simulink model "abslut125_fixpt16"  (R2021b)
(part 3 of 8)

  ROM6 : hdlBasic/ROM  depth=7874  initVector=[1,0,0,0,0,1,0,1,1,1,1,1,1,0,0,1,1,0,0,1,1,1,0,0,1,1,1,0,0,0,0,1,1,0,0,0,0,0,1,1,0,0,0,1,1,0,1,1,0,0,0,1,1,1,0,1,1,0,0,0,1,1,1,0,0,1,1,1,0,0,1,1,1,0,0,1,1,1,1,0,0,1,1,1,0,0,1,1,1,0,0,0,0,1,1,1,0,0,0,1,1,0,0,0,1,0,0,1,1,0,0,0,1,1,0,0,0,1,1,1,0,1,1,0,0,0,1,1,0,0,0,1,1,1,0,0,1,1,1,0,0,1,1,1,0,0,1,1,1,0,0,1,1,1,1,0,0,1,1,1,0,0,1,1,1,0,0,1,1,1,0,1,0,0,1,1,1,0,0,1,1,1,0,0,1,1,1,0,0,0,0,0,0,1,1,0,0,0,1,1,0,0,0,1,1,0,0,0,1,1,0,0,1,1,0,0,0,1,1,0,0,0,1,1,0,0,0,1,1,1,0,0,1,1,1,0,0,1,1,0,0,0,1,1,0,0,0,1,1,1,0,0,1,0,1,1,0,0,1,1,1,0,0,1,1,1,0,0,1,1,1,0,0,1,1,1,1,1,0,0,0,1,1,0,0,1,1,1,0,0,1,1,1,0,0,1,1,1,0,0,1,1,0,0,1,1,0,0,0,1,1,0,0,0,1,1,0,0,0,1,1,0,0,0,1,1,0,0,1,1,1,0,0,1,1,0,0,0,1,1,0,0,0,1,1,0,0,0,1,1,1,1,0,0,1,1,0,0,1,1,1,0,0,1,1,0,0,0,1,1,0,0,0,1,1,1,0,0,0,0,1,1,0,0,0,1,1,0,0,1,1,1,0,0,1,1,1,0,0,1,1,1,0,0,1,1,0,0,1,1,0,0,1,1,0,0,0,1,1,0,0,1,1,1,0,0,1,1,1,0,0,1,1,1,0,0,1,1,0,0,1,1,1,0,0,1,1,0,0,0,1,1,0,0,1,1,1,0,0,1,1,1,0,0,0,0,1,1,0,0,1,1,0,0,1,1,1,0,0,1,1,0,0,0,1,1,0,0,0,1,1,0,0,0,1,1,1,1,0,0,1,1,1,0,0,1,1,0,0,1,1,1,0,0,1,1,0,0,0,1,1,0,0,0,1,1,0,0,1,1,0,0,1,1,0,0,1,1,0,0,0,1,1,0,0,1,1,1,0,0,1,1,0,0,0,1,1,1,0,0,1,1,0,0,1,1,1,0,0,1,1,0,0,1,1,0,0,0,1,1,0,0,1,1,1,0,0,1,1,1,0,0,1,1,1,1,0,0,1,1,0,0,1,1,0,0,0,1,1,0,0,1,1,0,0,0,1,1,0,0,1,1,1,0,0,1,1,1,0,0,0,0,1,1,1,0,0,1,1,0,0,1,1,0,0,1,1,1,0,0,1,1,0,0,0,1,1,0,0,0,1,1,0,0,0,1,0,0,1,1,0,0,1,1,0,0,0,1,1,0,0,1,1,0,0,1,1,1,0,0,1,1,0,0,0,1,1,0,0,0,1,1,0,0,0,1,1,0,0,1,1,0,0,1,1,0,0,1,1,1,0,0,1,1,0,0,1,1,1,0,0,1,1,0,0,0,1,1,0,0,0,0,1,1,0,0,1,1,0,0,0,1,1,0,0,1,1,0,0,1,1,0,0,0,1,1,0,0,1,1,1,0,0,1,1,1,0,0,1,1,0,1,1,0,0,1,1,0,0,1,1,0,0,1,1,1,0,0,1,1,0,0,1,1,0,0,0,1,1,0,0,1,1,1,0,0,1,1,1,0,1,1,0,0,0,1,1,0,0,1,1,0,0,1,1,0,0,1,1,0,0,0,1,1,0,0,1,1,0,0,0,1,1,0,0,1,1,1,0,0,0,1,1,0,0,1,1,0,0,1,1,0,0,1,1,1,0,0,1,1,0,0,1,1,0,0,1,1,1,0,0,1,1,0,0,0,1,1,0,0,0,1,1,1,1,0,0,1,1,0,0,1,1,0,0,1,1,0,0,1,1,0,0,0,1,1,0,0,1,1,0,0,1,1,1,0,0,1,1,0,0,0,1,1,0,0,1,0,0,1,1,1,0,0,1,1,0,0,1,1,0,0,1,1,0,0,1,1,0,0,1,1,1,0,0,1,1,0,0,1,1,1,0,0,1,1,1,0,0,1,1,0,0,1,1,0,0,1,1,0,0,1,1,0,0,1,1,1,0,0,1,1,0,0,1,1,0,0,1,1,0,0,0,1,1,0,0,1,1,1,0,0,1,1,1,1,0,0,1,1,0,0,1,1,0,0,1,1,0,0,1,1,0,0,1,1,0,0,1,1,1,0,0,1,1,0,0,1,1,0,0,0,1,1,0,0,1,1,1,0,0,1,0,0,1,1,0,0,1,1,0,0,1,1,0,0,1,1,0,0,1,1,0,0,1,1,0,0,1,1,0,0,0,1,1,0,0,1,1,0,0,0,1,1,0,0,0,1,0,0,1,1,0,0,1,1,0,0,1,1,0,0,1,1,0,0,1,1,1,0,0,1,1,0,0,1,1,0,0,1,1,0,0,1,1,1,0,0,1,1,0,0,0,1,1,0,0,0,1,1,0,0,1,1,0,0,1,1,0,0,1,1,0,0,1,1,0,0,1,1,0,0,1,1,0,0,0,1,1,0,0,1,1,0,0,1,1,1,0,0,1,1,0,0,0,0,0,1,1,0,0,1,1,0,0,1,1,0,0,1,1,0,0,1,1,0,0,1,1,0,0,1,1,0,0,1,1,0,0,1,1,1,0,0,1,1,0,0,1,1,1,0,0,1,1,0,0,1,1,0,0,1,1,0,0,1,1,0,0,1,1,0,0,1,1,0,0,1,1,0,0,1,1,0,0,1,1,0,0,1,1,0,0,1,1,0,0,0,1,1,0,0,1,1,1,0,0,1,1,0,0,1,1,0,0,1,1,0,0,1,1,0,0,1,1,0,0,1,1,0,0,1,1,0,0,1,1,0,0,0,1,1,0,0,1,1,0,0,1,1,0,0,0,1,1,0,0,0,0,1,1,0,0,1,1,0,0,1,1,0,0,1,1,0,0,1,1,0,0,1,1,0,0,1,1,0,0,1,1,0,0,1,1,0,0,1,1,0,0,0,1,1,0,0,1,1,0,0,0,1,1,0,1,1,0,0,1,1,0,0,1,1,0,0,1,1,0,0,1,1,0,0,1,1,0,0,1,1,0,0,1,1,0,0,1,1,0,0,1,1,0,0,1,1,0,0,1,1,1,0,0,1,1,0,0,0,1,1,0,0,1,1,0,0,1,1,0,0,1,1,0,0,1,1,0,0,1,1,0,0,1,1,0,0,1,1,0,0,1,1,0,0,1,1,0,0,1,1,0,0,1,1,0,0,1,1,1,0,0,1,0,1,1,0,0,1,1,0,0,1,1,0,0,1,1,0,0,1,0,0,1,1,0,0,1,1,0,0,1,1,0,0,1,1,0,0,1,1,0,0,1,1,0,0,1,1,1,0,0,1,1,0,0,1,1,1,0,1,1,0,0,1,1,0,0,1,1,0,1,1,0,0,1,1,0,0,1,1,0,0,1,1,0,0,1,1,0,0,1,1,0,0,1,1,0,0,1,1,0,0,1,1,0,0,1,1,0,0,0,1,1,0,0,0,1,1,0,0,1,1,0,1,1,0,0,1,1,0,0,1,1,0,0,1,1,0,0,1,1,0,0,1,1,0,0,1,1,0,0,1,1,0,0,1,1,0,0,1,1,0,0,1,1,0,0,1,1,0,0,0,1,0,1,1,0,0,1,0,0,1,1,0,0,1,1,0,0,1,1,0,0,1,1,0,0,1,1,0,0,1,1,0,0,1,1,0,0,1,1,0,0,1,1,0,0,1,1,0,0,1,1,0,0,1,1,0,0,1,1,0,0,1,1,0,1,1,0,0,1,1,0,0,1,1,0,0,1,1,0,0,1,1,0,0,1,1,0,0,1,1,0,0,1,1,0,0,1,0,0,1,1,0,0,1,1,0,0,1,1,0,0,1,1,0,0,1,1,1,0,0,0,1,0,0,1,1,0,0,1,1,0,0,1,1,0,0,1,1,0,0,1,1,0,0,1,1,0,0,1,1,0,0,1,1,0,1,1,0,0,1,1,0,0,1,1,0,0,1,1,0,0,1,1,0,0,1,1,0,0,1,1,0,1,0,0,1,1,0,0,1,1,0,0,1,1,0,0,1,1,0,0,1,1,0,0,1,1,0,0,1,1,0,0,1,0,0,1,1,0,0,1,1,0,0,1,1,0,0,1,1,0,0,1,1,0,0,1,1,0,0,1,1,0,0,1,0,0,1,1,0,0,1,1,0,0,1,1,0,0,1,1,0,0,1,1,0,0,1,1,0,0,1,1,0,0,1,0,0,1,1,0,0,1,1,0,0,1,1,0 ...(+11750 chars)]  distributed_mem=Block RAM  rst=off  init_reg=0  en=off  latency=1  gui_display_data_type=Boolean  arith_type=Boolean  n_bits=2  bin_pt=0  preci_type=Double  exp_width=8  frac_width=24  optimize=Area  use_rpm=on  simulation_type=fast_sim  XmcBlockStatus=1  maskContainerNames=tabcontainer1  block_type=sprom  block_config=sysgen:SPROM_config
  ROM7 : hdlBasic/ROM  depth=7874  initVector=[0,1,1,1,0,1,0,1,0,0,1,0,0,1,0,0,0,1,0,1,1,0,1,0,1,1,0,1,1,0,0,1,0,1,1,0,0,0,1,0,1,1,0,1,0,0,1,0,1,1,0,1,0,0,1,1,0,1,1,0,1,0,0,1,0,1,0,0,1,0,1,0,0,1,0,1,1,0,0,1,0,1,1,0,1,0,1,1,0,1,0,1,0,1,1,0,1,0,0,1,0,1,1,0,1,0,0,1,0,1,0,0,1,0,1,1,0,1,0,0,0,1,0,1,1,0,1,0,1,1,0,1,0,0,1,0,1,0,0,1,0,1,0,0,1,0,1,0,0,1,0,1,1,1,0,1,0,1,0,0,1,0,1,0,0,1,0,1,1,0,1,0,1,0,1,1,0,1,0,1,1,0,1,0,1,1,0,1,0,0,1,1,0,1,0,1,0,0,1,0,1,0,0,1,0,1,0,0,1,0,1,0,1,0,1,1,0,1,0,1,0,0,1,0,1,1,0,1,0,0,1,0,1,1,0,1,0,1,0,1,1,0,1,0,1,1,0,1,0,0,1,0,1,0,1,0,1,0,1,1,0,1,0,1,0,0,1,0,1,0,0,1,0,1,1,0,1,0,1,1,0,1,0,1,0,1,1,0,1,0,1,1,0,1,0,1,1,0,1,0,1,0,1,0,1,0,1,1,0,1,0,1,0,0,1,0,1,0,0,1,0,1,0,0,1,0,1,0,1,1,0,1,0,1,0,1,1,0,1,0,1,0,0,1,0,1,1,0,1,0,0,0,1,0,1,0,1,0,1,0,0,1,0,1,0,1,1,0,1,0,1,1,0,1,0,0,1,0,1,0,1,0,1,1,0,1,0,1,0,1,1,0,1,0,1,0,0,1,0,1,0,0,1,0,1,1,0,0,1,0,1,0,1,0,1,0,0,1,0,1,0,1,1,0,1,0,1,0,0,1,0,1,1,0,1,0,1,0,1,0,1,1,0,1,0,1,0,1,0,0,1,0,1,0,1,1,0,1,0,1,1,0,1,0,0,0,1,0,1,0,1,0,1,0,1,1,0,1,0,1,0,1,0,0,1,0,1,0,0,1,0,1,0,0,1,0,1,0,1,0,1,0,0,1,0,1,0,1,0,1,0,0,1,0,1,0,1,1,0,1,0,1,1,0,1,0,1,1,1,0,1,0,1,0,1,0,1,0,1,1,0,1,0,1,0,1,0,0,1,0,1,0,1,1,0,1,0,0,1,0,1,0,1,0,1,0,0,1,0,1,0,1,0,1,0,1,1,0,1,0,1,0,1,1,0,1,0,1,0,0,1,0,1,1,0,0,1,0,1,0,1,0,1,0,1,0,0,1,0,1,0,1,0,1,0,0,1,0,1,0,1,1,0,1,0,1,1,0,1,0,1,0,1,0,0,1,0,1,0,1,0,1,0,1,0,1,1,0,1,0,1,0,1,0,0,1,0,1,0,0,1,0,1,0,0,1,1,0,1,0,1,0,1,0,1,0,0,1,0,1,0,1,0,1,0,1,0,0,1,0,1,0,1,1,0,1,0,1,0,0,1,0,1,1,0,1,0,1,0,1,0,1,0,1,0,1,0,1,0,0,1,0,1,0,1,0,1,0,0,1,0,1,0,1,1,0,1,0,1,1,0,0,1,0,1,0,1,0,1,0,0,1,0,1,0,1,0,1,0,1,0,1,1,0,1,0,1,0,1,0,0,1,0,1,0,0,1,0,1,1,0,1,0,1,0,1,0,1,0,1,0,1,0,1,0,0,1,0,1,0,1,0,1,0,1,0,0,1,0,1,0,1,1,0,1,0,1,1,0,1,1,0,1,0,0,1,0,1,0,1,0,1,0,1,0,1,0,1,0,1,0,0,1,0,1,0,1,0,1,0,0,1,0,1,0,1,1,0,1,0,0,1,0,1,0,1,0,1,0,1,0,1,0,1,1,0,1,0,1,0,1,0,1,0,1,0,1,1,0,1,0,1,0,1,0,0,1,0,1,0,0,1,0,1,0,1,0,1,0,1,0,1,0,1,0,1,0,1,0,1,0,1,0,0,1,0,1,0,1,0,1,0,1,0,0,1,0,1,0,1,1,0,1,0,1,1,0,1,0,1,1,0,1,0,1,0,1,0,1,0,1,0,1,0,1,0,1,0,1,0,1,0,0,1,0,1,0,1,0,1,0,0,1,0,1,0,0,1,0,1,0,1,0,1,0,1,0,1,0,1,0,1,0,1,0,1,0,0,1,0,1,0,1,0,1,0,1,0,1,0,1,1,0,1,0,1,0,1,0,0,1,0,1,1,0,0,1,0,1,0,1,0,1,0,1,0,1,0,1,0,1,0,1,0,1,0,1,0,1,0,0,1,0,1,0,1,0,1,0,1,0,0,1,0,1,0,1,1,0,1,0,0,1,0,1,0,1,0,1,0,1,0,1,0,1,0,1,0,1,0,1,0,1,0,1,0,1,0,1,0,1,0,0,1,0,1,0,1,0,1,0,0,1,0,1,0,0,1,1,0,1,0,1,0,1,0,1,0,1,0,1,0,1,0,1,0,1,1,0,1,0,1,0,1,0,1,0,1,0,1,0,1,0,1,0,0,1,0,1,0,1,0,0,1,0,1,1,0,1,0,1,0,1,0,1,0,1,0,1,0,1,0,1,0,1,0,1,0,1,0,1,0,1,0,1,1,0,1,0,1,0,1,0,1,0,1,0,0,1,0,1,0,1,1,0,1,0,1,0,1,0,1,0,1,0,1,0,1,0,1,0,1,0,1,0,1,0,1,0,1,0,1,0,1,0,1,0,1,0,1,0,0,1,0,1,0,1,0,1,0,0,1,0,1,0,1,0,1,0,1,0,1,0,1,0,1,0,1,0,1,0,1,0,1,0,1,0,1,0,1,0,1,0,1,0,1,0,1,0,1,0,1,0,1,0,1,0,0,1,0,1,0,1,1,0,1,0,1,0,1,0,1,0,1,0,1,0,1,0,1,0,1,0,1,0,1,0,1,0,1,0,1,0,1,0,1,0,1,0,0,1,0,1,0,1,0,1,0,1,0,1,0,0,1,0,1,0,0,0,1,0,1,0,1,0,1,0,1,0,1,0,1,0,1,0,1,0,1,0,1,0,1,0,1,0,1,0,1,0,1,0,1,0,1,0,1,0,1,0,0,1,0,1,0,1,0,1,0,0,1,0,0,1,0,1,0,1,0,1,0,1,0,1,0,1,0,1,0,1,0,1,0,1,0,1,0,1,0,1,0,1,0,1,0,1,0,1,0,1,0,1,0,1,0,1,0,1,0,0,1,0,1,0,1,1,0,1,0,1,0,1,0,1,0,1,0,1,0,1,0,1,0,1,0,1,0,1,0,1,0,1,0,1,0,1,0,1,0,1,0,1,0,1,0,1,0,1,0,1,0,1,0,1,0,1,0,0,1,0,1,0,1,0,1,0,1,0,1,0,1,0,1,0,1,0,1,0,1,1,0,1,0,1,0,1,0,1,0,1,0,1,0,1,0,1,0,1,0,1,0,1,0,1,0,1,0,0,1,0,1,0,1,0,1,0,0,0,1,0,1,0,1,0,1,0,1,0,1,1,0,1,0,1,0,1,0,1,0,1,0,1,0,1,0,1,0,1,0,1,0,1,0,1,0,1,0,1,0,1,0,1,0,1,0,1,0,1,0,0,1,0,1,0,0,1,0,1,0,1,0,1,1,0,1,0,1,0,1,0,1,0,1,0,1,0,1,0,1,0,1,0,1,0,1,0,1,0,1,0,1,0,1,0,1,0,1,0,1,0,1,0,1,0,1,0,1,0,1,0,0,1,0,1,0,1,0,0,1,0,1,0,1,0,1,0,1,0,1,0,1,0,1,0,1,0,1,0,1,0,1,0,1,0,1,0,1,0,1,0,1,0,1,0,1,0,1,0,1,0,1,0,1,0,1,0,1,0,1,0,1,0,1,0,0,1,0,1,0,1,0,1,0,1,0,1,0,1,0,1,0,1,0,1,0,1,0,1,0,1,0,1,0,1,0,1,0,1,1,0,1,0,1,0,1,0,1,0,1,0,1,0,1,0,1,0,1,0,0,1,0,0,1,1,0,1,0,1,0,1,0,1,0,1,0,1,0,1,0,1,0,1,0,1,0,1,0,1,0,1,0,1,0,1,0,0,1,0,1,0,1,0,1,0,1,0,1,0,1,0,1,0,1,0,1,0,1,0,1,0,1,0,0,0,1,0,1,0,1,0,1,0,1,0,1,0,1,0,1,0,1,0,1,0,1,0,1,0,1,0,1,0,1,0,0,1,0,1,0,1,0,1,0,1,0,1,0,1,0,1,0,1,0,1,0,1,0,1,0,1,0,1,0,1,0,0,1,0,1,0,1,0,1,0,1,0,1,0,1,0,1,0,1,0,1,0,1,0,1,0,1,0,1,0,1,0,0,1,0,1,0,1,0,1,0,1,0,1,0,1 ...(+11750 chars)]  distributed_mem=Block RAM  rst=off  init_reg=0  en=off  latency=1  gui_display_data_type=Boolean  arith_type=Boolean  n_bits=2  bin_pt=0  preci_type=Double  exp_width=8  frac_width=24  optimize=Area  use_rpm=on  simulation_type=fast_sim  XmcBlockStatus=1  maskContainerNames=tabcontainer1  block_type=sprom  block_config=sysgen:SPROM_config
  ROM8 : hdlBasic/ROM  depth=7874  initVector=[1,1,0,0,0,1,0,1,1,0,1,1,0,0,1,1,0,0,1,1,0,0,0,1,1,0,0,1,1,1,0,0,1,1,0,0,1,0,0,1,1,0,0,1,1,0,0,1,1,0,0,1,1,0,0,1,1,1,0,0,1,1,0,0,1,1,1,0,0,1,1,1,0,0,1,1,0,0,0,0,1,1,0,0,0,1,1,0,0,1,1,1,1,1,0,0,1,1,0,0,1,1,0,0,1,1,0,0,1,1,1,0,0,1,1,0,0,1,1,0,0,0,1,1,0,0,0,1,1,0,0,1,1,0,0,1,1,1,0,0,0,1,1,0,0,0,1,1,0,0,1,1,0,0,0,0,1,1,1,0,0,1,1,1,0,0,1,1,0,0,1,0,1,1,1,0,0,1,1,1,0,0,1,1,1,0,0,1,1,0,1,0,0,0,1,1,1,0,0,0,1,1,0,0,1,1,1,0,1,1,0,0,1,1,1,0,0,0,1,1,1,0,0,1,1,0,0,1,1,0,0,1,1,0,0,0,0,1,1,1,0,0,1,1,1,0,0,1,1,0,0,1,1,0,0,0,1,1,1,0,0,0,1,1,1,0,0,0,1,1,0,0,1,1,0,0,1,1,1,0,0,0,0,1,1,1,0,0,0,1,1,0,0,0,1,1,0,0,1,1,0,0,0,0,1,1,1,0,0,0,0,1,1,0,0,0,1,1,0,0,0,1,1,0,0,1,1,1,1,0,0,0,0,1,1,1,0,0,0,1,1,1,0,0,1,1,0,0,0,1,0,0,0,0,0,0,1,1,1,1,0,0,0,1,1,1,0,0,0,1,1,0,0,1,1,0,0,1,0,1,1,1,1,0,0,0,0,1,1,1,0,0,0,0,1,1,0,0,0,1,1,0,0,1,1,0,1,0,0,0,0,1,1,1,1,1,0,0,0,1,1,1,0,0,0,1,1,1,0,0,1,1,0,0,1,1,1,1,1,1,1,0,0,0,0,1,1,1,1,0,0,0,1,1,1,0,0,1,1,1,0,0,1,1,0,0,0,0,0,0,0,1,1,1,1,0,0,0,0,1,1,1,1,0,0,1,1,1,0,0,0,1,1,0,0,1,1,1,1,1,1,1,0,0,0,0,0,1,1,1,1,0,0,0,1,1,1,0,0,0,1,1,0,0,0,1,1,0,0,0,0,0,0,0,1,1,1,1,1,0,0,0,0,1,1,1,1,0,0,0,1,1,1,0,0,1,1,0,0,1,1,1,1,1,1,1,0,0,0,0,0,0,1,1,1,1,0,0,0,0,1,1,1,0,0,0,1,1,1,0,0,1,1,0,0,0,0,0,0,0,1,1,1,1,1,1,0,0,0,0,0,1,1,1,1,0,0,0,1,1,1,0,0,0,1,1,0,0,1,1,1,1,1,1,0,0,0,0,0,0,0,1,1,1,1,1,0,0,0,0,1,1,1,1,0,0,0,1,1,0,0,0,1,1,0,0,0,0,1,1,1,1,1,1,1,1,0,0,0,0,0,0,1,1,1,1,1,0,0,0,1,1,1,0,0,0,1,1,1,0,0,1,1,0,0,0,0,0,0,0,0,0,0,1,1,1,1,1,1,0,0,0,0,0,1,1,1,1,0,0,0,1,1,1,0,0,1,1,1,0,0,1,1,1,1,1,1,1,1,1,0,0,0,0,0,0,0,1,1,1,1,1,0,0,0,0,1,1,1,1,0,0,0,1,1,0,0,1,1,0,0,0,0,0,0,0,0,1,1,1,1,1,1,1,1,0,0,0,0,0,0,1,1,1,1,1,0,0,0,1,1,1,0,0,0,1,1,0,0,1,1,1,1,1,0,0,0,0,0,0,0,0,0,0,1,1,1,1,1,1,1,0,0,0,0,0,1,1,1,1,0,0,0,1,1,1,0,0,1,1,0,1,1,1,1,1,1,1,1,1,1,1,1,1,0,0,0,0,0,0,0,0,1,1,1,1,1,0,0,0,0,1,1,1,1,0,0,0,1,1,0,0,1,0,0,0,0,0,0,0,0,0,0,1,1,1,1,1,1,1,1,1,1,0,0,0,0,0,0,1,1,1,1,1,0,0,0,1,1,1,0,0,0,1,1,0,1,1,1,1,0,0,0,0,0,0,0,0,0,0,0,0,0,0,0,1,1,1,1,1,1,1,0,0,0,0,0,1,1,1,1,0,0,0,1,1,0,0,0,1,1,1,1,1,1,1,1,1,1,1,1,1,1,1,1,1,1,0,0,0,0,0,0,0,0,0,1,1,1,1,1,0,0,0,0,0,1,1,1,0,0,1,1,0,0,0,0,0,0,0,0,0,0,0,0,0,0,1,1,1,1,1,1,1,1,1,1,1,1,1,0,0,0,0,0,0,0,1,1,1,1,0,0,0,1,1,1,0,0,1,1,0,0,0,0,0,0,0,0,0,0,0,0,0,0,0,0,0,0,0,0,0,0,0,1,1,1,1,1,1,1,1,0,0,0,0,0,1,1,1,1,0,0,0,1,1,0,0,1,1,1,1,1,1,1,1,1,1,1,1,1,1,1,1,1,1,1,0,0,0,0,0,0,0,0,0,0,0,0,1,1,1,1,1,1,0,0,0,0,1,1,1,0,0,1,1,1,1,1,1,1,1,1,1,1,1,1,1,1,1,1,1,1,1,1,1,1,1,1,1,1,1,1,1,1,0,0,0,0,0,0,0,0,1,1,1,1,0,0,0,1,1,1,0,0,0,0,0,0,0,0,0,0,0,0,0,0,0,0,0,0,0,0,0,0,0,0,0,0,0,0,1,1,1,1,1,1,1,1,1,1,0,0,0,0,0,0,1,1,1,0,0,0,1,1,0,0,0,0,0,0,0,0,0,0,0,0,0,0,0,0,0,0,0,0,0,0,0,0,0,0,0,0,0,0,0,0,0,0,0,0,1,1,1,1,1,1,0,0,0,0,1,1,0,0,1,1,1,1,1,1,1,1,1,1,1,1,1,1,1,1,1,1,1,1,1,1,1,1,1,1,1,1,1,1,1,1,1,1,0,0,0,0,0,0,0,0,0,1,1,1,1,0,0,0,1,1,0,1,1,1,1,1,1,1,1,1,1,1,1,1,1,1,1,1,1,1,1,1,1,1,1,1,1,1,1,1,1,1,1,1,1,1,1,1,1,1,1,1,0,0,0,0,0,0,1,1,1,0,0,1,1,1,1,1,1,1,1,1,1,0,0,0,0,0,0,0,0,0,0,0,0,0,0,0,0,0,0,0,0,0,0,0,0,0,0,0,0,0,0,0,1,1,1,1,1,1,1,0,0,0,0,1,1,0,1,1,0,0,0,0,0,0,0,0,0,0,0,0,0,0,0,0,0,0,0,0,0,0,0,0,0,0,0,0,0,0,0,0,0,0,0,0,0,0,0,0,0,0,0,0,0,1,1,1,1,0,0,0,1,0,0,0,0,0,0,0,0,0,0,0,0,0,0,0,0,0,0,1,1,1,1,1,1,1,1,1,1,1,1,1,1,1,1,1,1,1,1,1,1,1,1,1,1,1,1,0,0,0,0,0,0,1,1,1,0,0,0,0,0,0,0,0,0,0,0,0,0,1,1,1,1,1,1,1,1,1,1,1,1,1,1,1,1,1,1,1,1,1,1,1,1,1,1,1,1,1,1,1,1,1,1,1,1,1,1,1,1,0,0,0,1,1,0,0,0,0,0,0,0,0,1,1,1,1,1,1,1,1,1,1,1,1,1,1,1,1,1,1,1,0,0,0,0,0,0,0,0,0,0,0,0,0,0,0,0,0,0,0,0,0,0,0,0,0,1,1,1,1,0,0,0,0,0,0,0,1,1,1,1,1,1,1,1,1,1,1,1,1,1,1,1,1,0,0,0,0,0,0,0,0,0,0,0,0,0,0,0,0,0,0,0,0,0,0,0,0,0,0,0,0,0,0,0,0,0,0,0,1,1,0,0,0,1,1,1,1,1,1,1,1,1,1,1,1,1,1,1,1,0,0,0,0,0,0,0,0,0,0,0,0,0,0,0,0,0,0,1,1,1,1,1,1,1,1,1,1,1,1,1,1,1,1,1,1,1,1,0,0,0,0,0,1,1,1,1,1,1,1,1,1,1,1,1,1,1,1,0,0,0,0,0,0,0,0,0,0,0,0,0,0,0,0,0,1,1,1,1,1,1,1,1,1,1,1,1,1,1,1,1,1,1,1,1,1,1,1,1,1,1,1,0,1,1,1,1,1,1,1,1,1,1,1,1,1,1,1,0,0,0,0,0,0,0,0,0,0,0,0,0,0,0,0,1,1,1,1,1,1,1,1,1,1,1,1,1,1,1,1,0,0,0,0,0,0,0,0,0,0,0,0,0,0,0,1,1,1,1,1,1,1,1,1,1,1,1,1,1,1,0,0,0,0,0,0,0,0,0,0,0,0,0,0,0,0,1,1,1,1,1,1,1,1,1,1,1,1,1,1 ...(+11750 chars)]  distributed_mem=Block RAM  rst=off  init_reg=0  en=off  latency=1  gui_display_data_type=Boolean  arith_type=Boolean  n_bits=2  bin_pt=0  preci_type=Double  exp_width=8  frac_width=24  optimize=Area  use_rpm=on  simulation_type=fast_sim  XmcBlockStatus=1  maskContainerNames=tabcontainer1  block_type=sprom  block_config=sysgen:SPROM_config
  ROM9 : hdlBasic/ROM  depth=7874  initVector=[0,1,0,0,1,0,1,0,1,0,0,1,0,1,0,1,0,1,0,1,0,0,1,0,1,0,1,1,0,1,0,1,0,1,0,1,1,0,1,0,1,0,1,0,1,0,1,0,1,0,1,0,1,0,1,0,0,1,0,1,0,1,0,1,0,1,1,0,1,0,0,1,0,1,0,1,0,1,0,1,0,1,0,1,1,0,1,0,1,0,1,0,1,1,0,1,0,1,0,1,0,1,0,1,0,1,0,1,0,0,1,0,1,0,1,0,1,0,1,0,1,1,0,1,0,1,1,0,1,0,1,0,1,0,1,0,0,1,0,0,1,0,1,0,0,1,0,1,0,1,0,1,0,0,0,1,0,1,1,0,1,0,1,1,0,1,0,1,0,1,0,1,0,1,1,0,1,0,0,1,0,1,0,1,1,0,1,0,1,0,1,0,0,1,0,0,1,0,1,1,0,1,0,1,0,1,1,0,0,1,1,1,0,1,1,0,1,1,0,1,1,0,1,0,1,0,1,0,1,0,1,0,1,0,0,1,1,0,1,1,0,1,0,0,1,0,1,0,1,0,1,0,1,0,1,1,0,0,1,0,0,1,0,0,1,0,1,1,0,1,0,1,0,1,0,1,0,0,1,0,0,1,1,0,1,1,0,1,1,0,1,0,1,1,0,1,0,1,0,1,0,0,1,1,0,0,1,0,0,1,1,0,1,0,0,1,0,1,0,0,1,0,1,0,1,0,0,1,1,0,0,1,1,0,0,1,0,0,1,0,0,1,0,1,0,1,0,0,1,0,0,0,0,0,1,1,0,0,1,1,0,1,1,0,1,1,0,1,1,0,1,0,1,0,1,0,1,0,1,0,0,1,1,0,0,1,1,0,0,1,0,0,1,1,0,1,0,0,1,0,1,0,1,0,1,0,1,0,0,1,1,0,0,0,1,1,0,1,1,0,0,1,0,0,1,0,1,1,0,1,0,1,0,1,0,0,0,0,1,1,1,0,0,1,1,0,0,1,1,0,1,1,0,1,1,0,1,0,0,1,0,1,0,1,0,0,0,0,1,1,1,0,0,1,1,0,0,1,1,0,0,1,1,0,1,0,0,1,0,1,1,0,1,0,1,0,0,0,0,1,1,1,0,0,1,1,1,0,0,1,1,0,1,1,0,0,1,0,0,1,0,1,0,1,1,0,1,1,0,0,0,1,1,1,0,0,1,1,1,0,0,1,1,0,0,1,1,0,1,1,0,1,1,0,1,0,1,0,1,0,1,0,0,1,1,1,0,0,0,1,1,1,0,0,1,1,0,0,1,1,0,0,1,0,0,1,0,0,1,0,1,0,1,0,1,0,1,1,1,1,0,0,0,1,1,1,0,0,1,1,1,0,0,1,1,0,1,1,0,0,1,0,1,1,0,1,0,1,0,1,1,1,1,1,0,0,0,0,1,1,1,0,0,1,1,1,0,0,1,1,0,0,1,1,0,1,1,0,1,0,0,1,0,1,0,1,1,1,0,0,0,0,0,1,1,1,0,0,0,1,1,1,0,0,1,1,1,0,0,1,0,0,1,0,0,1,0,1,1,0,1,0,1,0,0,0,0,0,0,1,1,1,1,0,0,0,1,1,1,0,0,0,1,1,0,0,1,1,0,0,1,0,0,1,0,1,0,0,1,0,1,0,0,0,0,1,1,1,1,1,0,0,0,1,1,1,1,0,0,0,1,1,0,0,1,1,0,0,1,1,0,1,1,0,1,0,1,0,1,0,1,1,1,1,1,1,1,0,0,0,0,1,1,1,1,0,0,0,1,1,1,0,0,0,1,1,0,0,1,0,0,1,0,0,1,0,1,0,1,0,1,1,1,1,0,0,0,0,0,0,1,1,1,1,0,0,0,0,1,1,1,0,0,0,1,1,0,0,1,1,0,0,1,0,1,1,0,1,0,1,0,0,0,0,0,0,0,0,1,1,1,1,1,1,0,0,0,0,1,1,1,1,0,0,0,1,1,0,0,1,1,0,0,1,1,0,1,1,0,1,0,1,0,0,1,1,1,1,1,1,1,1,1,0,0,0,0,0,0,1,1,1,1,0,0,0,0,1,1,0,0,0,1,1,0,0,1,0,0,1,0,0,1,0,1,0,1,1,1,1,0,0,0,0,0,0,0,0,0,1,1,1,1,1,1,0,0,0,0,1,1,1,0,0,0,1,1,0,0,1,1,0,0,1,0,1,0,0,1,0,0,0,0,0,0,0,0,0,1,1,1,1,1,1,1,1,1,0,0,0,0,0,1,1,1,1,0,0,0,1,1,0,0,0,1,1,0,1,1,0,1,0,1,0,1,1,1,1,1,1,1,1,1,1,1,1,1,0,0,0,0,0,0,0,0,1,1,1,1,1,0,0,0,0,1,1,1,0,0,1,1,0,0,1,0,0,1,0,1,0,1,0,0,0,0,0,0,0,0,0,0,0,0,0,0,0,1,1,1,1,1,1,1,1,0,0,0,0,0,1,1,1,0,0,0,1,1,0,0,1,1,0,1,1,0,1,0,1,1,1,1,1,1,1,1,1,1,1,1,1,1,1,1,1,1,1,1,0,0,0,0,0,0,0,1,1,1,1,1,0,0,0,1,1,1,0,0,1,1,0,1,1,0,1,0,1,0,0,0,0,0,0,0,0,0,0,0,0,0,0,0,0,0,0,0,0,0,0,0,1,1,1,1,1,1,0,0,0,0,0,1,1,1,0,0,1,1,0,0,1,0,0,1,0,1,1,1,1,1,1,1,1,1,1,1,1,1,1,1,1,1,1,1,1,1,1,1,1,1,1,1,0,0,0,0,0,0,1,1,1,1,0,0,0,1,1,1,0,1,1,0,1,1,0,1,0,0,0,0,0,0,0,0,0,0,0,0,0,0,0,0,0,0,0,0,0,0,0,0,0,0,0,0,0,0,1,1,1,1,1,1,0,0,0,1,1,1,0,0,1,1,0,1,0,1,0,1,1,1,1,1,1,1,1,1,1,1,1,1,1,1,1,1,1,1,1,1,1,1,1,1,1,1,1,1,1,1,1,1,0,0,0,0,0,1,1,1,1,0,0,1,1,0,0,1,0,1,0,1,1,1,1,1,0,0,0,0,0,0,0,0,0,0,0,0,0,0,0,0,0,0,0,0,0,0,0,0,0,0,0,0,0,0,0,1,1,1,1,1,0,0,0,1,1,1,0,1,1,0,1,0,0,0,0,0,0,0,0,0,0,1,1,1,1,1,1,1,1,1,1,1,1,1,1,1,1,1,1,1,1,1,1,1,1,1,1,1,1,1,1,1,0,0,0,0,1,1,1,0,0,1,1,0,1,0,0,0,1,1,1,1,1,1,1,1,1,1,1,1,0,0,0,0,0,0,0,0,0,0,0,0,0,0,0,0,0,0,0,0,0,0,0,0,0,0,0,0,0,1,1,1,1,0,0,1,1,0,0,1,0,1,1,1,1,1,1,1,0,0,0,0,0,0,0,0,0,0,0,1,1,1,1,1,1,1,1,1,1,1,1,1,1,1,1,1,1,1,1,1,1,1,1,1,1,1,1,0,0,0,0,1,1,0,1,1,0,1,1,0,0,0,0,0,0,0,0,0,0,1,1,1,1,1,1,1,1,1,1,1,0,0,0,0,0,0,0,0,0,0,0,0,0,0,0,0,0,0,0,0,0,0,0,0,0,0,1,1,1,0,0,1,0,1,0,0,0,0,0,0,0,0,1,1,1,1,1,1,1,1,1,0,0,0,0,0,0,0,0,0,0,1,1,1,1,1,1,1,1,1,1,1,1,1,1,1,1,1,1,1,1,1,1,1,1,1,0,0,0,1,0,1,0,0,0,0,0,1,1,1,1,1,1,1,1,0,0,0,0,0,0,0,0,0,1,1,1,1,1,1,1,1,1,1,0,0,0,0,0,0,0,0,0,0,0,0,0,0,0,0,0,0,0,0,0,0,0,1,1,0,1,0,0,0,1,1,1,1,1,1,1,1,0,0,0,0,0,0,0,0,1,1,1,1,1,1,1,1,1,0,0,0,0,0,0,0,0,0,1,1,1,1,1,1,1,1,1,1,1,1,1,1,1,1,1,1,1,1,0,0,1,0,0,1,1,1,1,1,1,1,0,0,0,0,0,0,0,0,1,1,1,1,1,1,1,1,0,0,0,0,0,0,0,0,0,1,1,1,1,1,1,1,1,0,0,0,0,0,0,0,0,0,0,0,0,0,0,0,0,0,0,1,0,1,1,1,1,1,1,1,1,0,0,0,0,0,0,0,1,1,1,1,1,1,1,1,0,0,0,0,0,0,0,0,1,1,1,1,1,1,1,1,0,0,0,0,0,0,0,0,1,1,1,1,1,1,1,1,1,1,1,1,1,1,0,1,1,1,1,1,1,1,0,0,0,0,0,0,0,0,1,1,1,1,1,1,1,1,0,0,0,0,0,0,0,0,1,1,1,1,1,1,1,0,0,0,0,0,0,0 ...(+11750 chars)]  distributed_mem=Block RAM  rst=off  init_reg=0  en=off  latency=1  gui_display_data_type=Boolean  arith_type=Boolean  n_bits=2  bin_pt=0  preci_type=Double  exp_width=8  frac_width=24  optimize=Area  use_rpm=on  simulation_type=fast_sim  XmcBlockStatus=1  maskContainerNames=tabcontainer1  block_type=sprom  block_config=sysgen:SPROM_config
  Relational{98,101..106,111..118,120,122,129,131..140,142..151,153..162,164..173,175..208,210,238..239,250,253,258..262,264..273,275..284,286..295,297..302} (138 alike) : hdlBasic/Relational  mode=a>=b  op_type=Bool  en=off  latency=1  XmcBlockStatus=1  maskContainerNames=tabcontainer1  block_type=relational  block_config=sysgen:Relational_config
  Scaling : hdlBasic/Scale  scale_factor=-31  XmcBlockStatus=1  maskContainerNames=group1  block_type=scale  block_config=sysgen:Scale_config
  Slice : hdlBasic/Slice  nbits=7  boolean_output=off  mode=Lower Bit Location + Width  bit1=-1  base1=MSB of Input  bit0=0  base0=LSB of Input  XmcBlockStatus=1  maskContainerNames=group1  block_type=slice  block_config=sysgen:Slice_config
  Slice1 : hdlBasic/Slice  nbits=7  boolean_output=off  mode=Lower Bit Location + Width  bit1=-1  base1=MSB of Input  bit0=0  base0=LSB of Input  XmcBlockStatus=1  maskContainerNames=group1  block_type=slice  block_config=sysgen:Slice_config
  Slice2 : hdlBasic/Slice  nbits=21  boolean_output=off  mode=Two Bit Locations  bit1=-1  base1=MSB of Input  bit0=1  base0=LSB of Input  XmcBlockStatus=1  maskContainerNames=group1  block_type=slice  block_config=sysgen:Slice_config
  Slice3 : hdlBasic/Slice  nbits=21  boolean_output=off  mode=Two Bit Locations  bit1=-4  base1=MSB of Input  bit0=0  base0=LSB of Input  XmcBlockStatus=1  maskContainerNames=group1  block_type=slice  block_config=sysgen:Slice_config
  addsub{1..104,106..110} (109 alike) : hdlBasic/AddSub  mode=Addition  use_carryin=off  use_carryout=off  en=off  latency=1  precision=User Defined  arith_type="Signed  (2's comp)"  n_bits=32  bin_pt=0  quantization=Truncate  overflow=Wrap  use_behavioral_HDL=off  hw_selection=Fabric  pipelined=off  XmcBlockStatus=1  maskContainerNames=tabcontainer1  block_type=addsub  block_config=sysgen:Addsub_config
  adsbu105 : hdlBasic/AddSub  mode=Addition  use_carryin=off  use_carryout=off  en=off  latency=1  precision=User Defined  arith_type="Signed  (2's comp)"  n_bits=32  bin_pt=0  quantization=Truncate  overflow=Wrap  use_behavioral_HDL=off  hw_selection=Fabric  pipelined=off  XmcBlockStatus=1  maskContainerNames=tabcontainer1  block_type=addsub  block_config=sysgen:Addsub_config
  bool1 : hdlBasic/Relational  mode=a<b  op_type=Bool  en=off  latency=0  XmcBlockStatus=1  maskContainerNames=tabcontainer1  block_type=relational  block_config=sysgen:Relational_config
  logi_b0 : hdlBasic/Constant  const=-1.0000000000000000000000000000000000000000000000000000000  gui_display_data_type=Fixed-point  arith_type=Signed (2's comp)  n_bits=32  bin_pt=30  preci_type=Double  exp_width=8  frac_width=24  explicit_period=on  period=1  XmcBlockStatus=1  maskContainerNames=tabcontainer1  block_type=constant  block_config=sysgen:Constant_config
  logi_b1 : hdlBasic/Constant  const=-0.9838709677419354981964261241955682635307312011718750000  gui_display_data_type=Fixed-point  arith_type=Signed (2's comp)  n_bits=32  bin_pt=30  preci_type=Double  exp_width=8  frac_width=24  explicit_period=on  period=1  XmcBlockStatus=1  maskContainerNames=tabcontainer1  block_type=constant  block_config=sysgen:Constant_config
  logi_b10 : hdlBasic/Constant  const=-0.8387096774193547599196563169243745505809783935546875000  gui_display_data_type=Fixed-point  arith_type=Signed (2's comp)  n_bits=32  bin_pt=30  preci_type=Double  exp_width=8  frac_width=24  explicit_period=on  period=1  XmcBlockStatus=1  maskContainerNames=tabcontainer1  block_type=constant  block_config=sysgen:Constant_config
  logi_b100 : hdlBasic/Constant  const=0.6129032258064516236473195931466761976480484008789062500  gui_display_data_type=Fixed-point  arith_type=Signed (2's comp)  n_bits=32  bin_pt=30  preci_type=Double  exp_width=8  frac_width=24  explicit_period=on  period=1  XmcBlockStatus=1  maskContainerNames=tabcontainer1  block_type=constant  block_config=sysgen:Constant_config
  logi_b101 : hdlBasic/Constant  const=0.6290322580645161254508934689511079341173171997070312500  gui_display_data_type=Fixed-point  arith_type=Signed (2's comp)  n_bits=32  bin_pt=30  preci_type=Double  exp_width=8  frac_width=24  explicit_period=on  period=1  XmcBlockStatus=1  maskContainerNames=tabcontainer1  block_type=constant  block_config=sysgen:Constant_config
  logi_b102 : hdlBasic/Constant  const=0.6451612903225806272544673447555396705865859985351562500  gui_display_data_type=Fixed-point  arith_type=Signed (2's comp)  n_bits=32  bin_pt=30  preci_type=Double  exp_width=8  frac_width=24  explicit_period=on  period=1  XmcBlockStatus=1  maskContainerNames=tabcontainer1  block_type=constant  block_config=sysgen:Constant_config
  logi_b103 : hdlBasic/Constant  const=0.6612903225806451290580412205599714070558547973632812500  gui_display_data_type=Fixed-point  arith_type=Signed (2's comp)  n_bits=32  bin_pt=30  preci_type=Double  exp_width=8  frac_width=24  explicit_period=on  period=1  XmcBlockStatus=1  maskContainerNames=tabcontainer1  block_type=constant  block_config=sysgen:Constant_config
  logi_b104 : hdlBasic/Constant  const=0.6774193548387096308616150963644031435251235961914062500  gui_display_data_type=Fixed-point  arith_type=Signed (2's comp)  n_bits=32  bin_pt=30  preci_type=Double  exp_width=8  frac_width=24  explicit_period=on  period=1  XmcBlockStatus=1  maskContainerNames=tabcontainer1  block_type=constant  block_config=sysgen:Constant_config
  logi_b105 : hdlBasic/Constant  const=0.6935483870967741326651889721688348799943923950195312500  gui_display_data_type=Fixed-point  arith_type=Signed (2's comp)  n_bits=32  bin_pt=30  preci_type=Double  exp_width=8  frac_width=24  explicit_period=on  period=1  XmcBlockStatus=1  maskContainerNames=tabcontainer1  block_type=constant  block_config=sysgen:Constant_config
  logi_b106 : hdlBasic/Constant  const=0.7096774193548387454910653104889206588268280029296875000  gui_display_data_type=Fixed-point  arith_type=Signed (2's comp)  n_bits=32  bin_pt=30  preci_type=Double  exp_width=8  frac_width=24  explicit_period=on  period=1  XmcBlockStatus=1  maskContainerNames=tabcontainer1  block_type=constant  block_config=sysgen:Constant_config
  logi_b107 : hdlBasic/Constant  const=0.7258064516129032472946391862933523952960968017578125000  gui_display_data_type=Fixed-point  arith_type=Signed (2's comp)  n_bits=32  bin_pt=30  preci_type=Double  exp_width=8  frac_width=24  explicit_period=on  period=1  XmcBlockStatus=1  maskContainerNames=tabcontainer1  block_type=constant  block_config=sysgen:Constant_config
  logi_b108 : hdlBasic/Constant  const=0.7419354838709677490982130620977841317653656005859375000  gui_display_data_type=Fixed-point  arith_type=Signed (2's comp)  n_bits=32  bin_pt=30  preci_type=Double  exp_width=8  frac_width=24  explicit_period=on  period=1  XmcBlockStatus=1  maskContainerNames=tabcontainer1  block_type=constant  block_config=sysgen:Constant_config
  logi_b109 : hdlBasic/Constant  const=0.7580645161290322509017869379022158682346343994140625000  gui_display_data_type=Fixed-point  arith_type=Signed (2's comp)  n_bits=32  bin_pt=30  preci_type=Double  exp_width=8  frac_width=24  explicit_period=on  period=1  XmcBlockStatus=1  maskContainerNames=tabcontainer1  block_type=constant  block_config=sysgen:Constant_config
  logi_b11 : hdlBasic/Constant  const=-0.8225806451612902581160824411199428141117095947265625000  gui_display_data_type=Fixed-point  arith_type=Signed (2's comp)  n_bits=32  bin_pt=30  preci_type=Double  exp_width=8  frac_width=24  explicit_period=on  period=1  XmcBlockStatus=1  maskContainerNames=tabcontainer1  block_type=constant  block_config=sysgen:Constant_config
  logi_b110 : hdlBasic/Constant  const=0.7741935483870967527053608137066476047039031982421875000  gui_display_data_type=Fixed-point  arith_type=Signed (2's comp)  n_bits=32  bin_pt=30  preci_type=Double  exp_width=8  frac_width=24  explicit_period=on  period=1  XmcBlockStatus=1  maskContainerNames=tabcontainer1  block_type=constant  block_config=sysgen:Constant_config
  logi_b111 : hdlBasic/Constant  const=0.7903225806451612545089346895110793411731719970703125000  gui_display_data_type=Fixed-point  arith_type=Signed (2's comp)  n_bits=32  bin_pt=30  preci_type=Double  exp_width=8  frac_width=24  explicit_period=on  period=1  XmcBlockStatus=1  maskContainerNames=tabcontainer1  block_type=constant  block_config=sysgen:Constant_config
  logi_b112 : hdlBasic/Constant  const=0.8064516129032257563125085653155110776424407958984375000  gui_display_data_type=Fixed-point  arith_type=Signed (2's comp)  n_bits=32  bin_pt=30  preci_type=Double  exp_width=8  frac_width=24  explicit_period=on  period=1  XmcBlockStatus=1  maskContainerNames=tabcontainer1  block_type=constant  block_config=sysgen:Constant_config
  logi_b113 : hdlBasic/Constant  const=0.8225806451612902581160824411199428141117095947265625000  gui_display_data_type=Fixed-point  arith_type=Signed (2's comp)  n_bits=32  bin_pt=30  preci_type=Double  exp_width=8  frac_width=24  explicit_period=on  period=1  XmcBlockStatus=1  maskContainerNames=tabcontainer1  block_type=constant  block_config=sysgen:Constant_config
  logi_b114 : hdlBasic/Constant  const=0.8387096774193547599196563169243745505809783935546875000  gui_display_data_type=Fixed-point  arith_type=Signed (2's comp)  n_bits=32  bin_pt=30  preci_type=Double  exp_width=8  frac_width=24  explicit_period=on  period=1  XmcBlockStatus=1  maskContainerNames=tabcontainer1  block_type=constant  block_config=sysgen:Constant_config
  logi_b115 : hdlBasic/Constant  const=0.8548387096774193727455326552444603294134140014648437500  gui_display_data_type=Fixed-point  arith_type=Signed (2's comp)  n_bits=32  bin_pt=30  preci_type=Double  exp_width=8  frac_width=24  explicit_period=on  period=1  XmcBlockStatus=1  maskContainerNames=tabcontainer1  block_type=constant  block_config=sysgen:Constant_config
  logi_b116 : hdlBasic/Constant  const=0.8709677419354838745491065310488920658826828002929687500  gui_display_data_type=Fixed-point  arith_type=Signed (2's comp)  n_bits=32  bin_pt=30  preci_type=Double  exp_width=8  frac_width=24  explicit_period=on  period=1  XmcBlockStatus=1  maskContainerNames=tabcontainer1  block_type=constant  block_config=sysgen:Constant_config
  logi_b117 : hdlBasic/Constant  const=0.8870967741935483763526804068533238023519515991210937500  gui_display_data_type=Fixed-point  arith_type=Signed (2's comp)  n_bits=32  bin_pt=30  preci_type=Double  exp_width=8  frac_width=24  explicit_period=on  period=1  XmcBlockStatus=1  maskContainerNames=tabcontainer1  block_type=constant  block_config=sysgen:Constant_config
  logi_b118 : hdlBasic/Constant  const=0.9032258064516128781562542826577555388212203979492187500  gui_display_data_type=Fixed-point  arith_type=Signed (2's comp)  n_bits=32  bin_pt=30  preci_type=Double  exp_width=8  frac_width=24  explicit_period=on  period=1  XmcBlockStatus=1  maskContainerNames=tabcontainer1  block_type=constant  block_config=sysgen:Constant_config
  logi_b119 : hdlBasic/Constant  const=0.9193548387096773799598281584621872752904891967773437500  gui_display_data_type=Fixed-point  arith_type=Signed (2's comp)  n_bits=32  bin_pt=30  preci_type=Double  exp_width=8  frac_width=24  explicit_period=on  period=1  XmcBlockStatus=1  maskContainerNames=tabcontainer1  block_type=constant  block_config=sysgen:Constant_config
  logi_b12 : hdlBasic/Constant  const=-0.8064516129032257563125085653155110776424407958984375000  gui_display_data_type=Fixed-point  arith_type=Signed (2's comp)  n_bits=32  bin_pt=30  preci_type=Double  exp_width=8  frac_width=24  explicit_period=on  period=1  XmcBlockStatus=1  maskContainerNames=tabcontainer1  block_type=constant  block_config=sysgen:Constant_config
  logi_b120 : hdlBasic/Constant  const=0.9354838709677418817634020342666190117597579956054687500  gui_display_data_type=Fixed-point  arith_type=Signed (2's comp)  n_bits=32  bin_pt=30  preci_type=Double  exp_width=8  frac_width=24  explicit_period=on  period=1  XmcBlockStatus=1  maskContainerNames=tabcontainer1  block_type=constant  block_config=sysgen:Constant_config
  logi_b121 : hdlBasic/Constant  const=0.9516129032258063835669759100710507482290267944335937500  gui_display_data_type=Fixed-point  arith_type=Signed (2's comp)  n_bits=32  bin_pt=30  preci_type=Double  exp_width=8  frac_width=24  explicit_period=on  period=1  XmcBlockStatus=1  maskContainerNames=tabcontainer1  block_type=constant  block_config=sysgen:Constant_config
  logi_b122 : hdlBasic/Constant  const=0.9677419354838709963928522483911365270614624023437500000  gui_display_data_type=Fixed-point  arith_type=Signed (2's comp)  n_bits=32  bin_pt=30  preci_type=Double  exp_width=8  frac_width=24  explicit_period=on  period=1  XmcBlockStatus=1  maskContainerNames=tabcontainer1  block_type=constant  block_config=sysgen:Constant_config
  logi_b123 : hdlBasic/Constant  const=0.9838709677419354981964261241955682635307312011718750000  gui_display_data_type=Fixed-point  arith_type=Signed (2's comp)  n_bits=32  bin_pt=30  preci_type=Double  exp_width=8  frac_width=24  explicit_period=on  period=1  XmcBlockStatus=1  maskContainerNames=tabcontainer1  block_type=constant  block_config=sysgen:Constant_config
  logi_b124 : hdlBasic/Constant  const=1.0000000000000000000000000000000000000000000000000000000  gui_display_data_type=Fixed-point  arith_type=Signed (2's comp)  n_bits=32  bin_pt=30  preci_type=Double  exp_width=8  frac_width=24  explicit_period=on  period=1  XmcBlockStatus=1  maskContainerNames=tabcontainer1  block_type=constant  block_config=sysgen:Constant_config
  logi_b13 : hdlBasic/Constant  const=-0.7903225806451612545089346895110793411731719970703125000  gui_display_data_type=Fixed-point  arith_type=Signed (2's comp)  n_bits=32  bin_pt=30  preci_type=Double  exp_width=8  frac_width=24  explicit_period=on  period=1  XmcBlockStatus=1  maskContainerNames=tabcontainer1  block_type=constant  block_config=sysgen:Constant_config
  logi_b14 : hdlBasic/Constant  const=-0.7741935483870967527053608137066476047039031982421875000  gui_display_data_type=Fixed-point  arith_type=Signed (2's comp)  n_bits=32  bin_pt=30  preci_type=Double  exp_width=8  frac_width=24  explicit_period=on  period=1  XmcBlockStatus=1  maskContainerNames=tabcontainer1  block_type=constant  block_config=sysgen:Constant_config
  logi_b15 : hdlBasic/Constant  const=-0.7580645161290322509017869379022158682346343994140625000  gui_display_data_type=Fixed-point  arith_type=Signed (2's comp)  n_bits=32  bin_pt=30  preci_type=Double  exp_width=8  frac_width=24  explicit_period=on  period=1  XmcBlockStatus=1  maskContainerNames=tabcontainer1  block_type=constant  block_config=sysgen:Constant_config
  logi_b16 : hdlBasic/Constant  const=-0.7419354838709677490982130620977841317653656005859375000  gui_display_data_type=Fixed-point  arith_type=Signed (2's comp)  n_bits=32  bin_pt=30  preci_type=Double  exp_width=8  frac_width=24  explicit_period=on  period=1  XmcBlockStatus=1  maskContainerNames=tabcontainer1  block_type=constant  block_config=sysgen:Constant_config
  logi_b17 : hdlBasic/Constant  const=-0.7258064516129032472946391862933523952960968017578125000  gui_display_data_type=Fixed-point  arith_type=Signed (2's comp)  n_bits=32  bin_pt=30  preci_type=Double  exp_width=8  frac_width=24  explicit_period=on  period=1  XmcBlockStatus=1  maskContainerNames=tabcontainer1  block_type=constant  block_config=sysgen:Constant_config
  logi_b18 : hdlBasic/Constant  const=-0.7096774193548387454910653104889206588268280029296875000  gui_display_data_type=Fixed-point  arith_type=Signed (2's comp)  n_bits=32  bin_pt=30  preci_type=Double  exp_width=8  frac_width=24  explicit_period=on  period=1  XmcBlockStatus=1  maskContainerNames=tabcontainer1  block_type=constant  block_config=sysgen:Constant_config
  logi_b19 : hdlBasic/Constant  const=-0.6935483870967741326651889721688348799943923950195312500  gui_display_data_type=Fixed-point  arith_type=Signed (2's comp)  n_bits=32  bin_pt=30  preci_type=Double  exp_width=8  frac_width=24  explicit_period=on  period=1  XmcBlockStatus=1  maskContainerNames=tabcontainer1  block_type=constant  block_config=sysgen:Constant_config
  logi_b2 : hdlBasic/Constant  const=-0.9677419354838709963928522483911365270614624023437500000  gui_display_data_type=Fixed-point  arith_type=Signed (2's comp)  n_bits=32  bin_pt=30  preci_type=Double  exp_width=8  frac_width=24  explicit_period=on  period=1  XmcBlockStatus=1  maskContainerNames=tabcontainer1  block_type=constant  block_config=sysgen:Constant_config
  logi_b20 : hdlBasic/Constant  const=-0.6774193548387096308616150963644031435251235961914062500  gui_display_data_type=Fixed-point  arith_type=Signed (2's comp)  n_bits=32  bin_pt=30  preci_type=Double  exp_width=8  frac_width=24  explicit_period=on  period=1  XmcBlockStatus=1  maskContainerNames=tabcontainer1  block_type=constant  block_config=sysgen:Constant_config
  logi_b21 : hdlBasic/Constant  const=-0.6612903225806451290580412205599714070558547973632812500  gui_display_data_type=Fixed-point  arith_type=Signed (2's comp)  n_bits=32  bin_pt=30  preci_type=Double  exp_width=8  frac_width=24  explicit_period=on  period=1  XmcBlockStatus=1  maskContainerNames=tabcontainer1  block_type=constant  block_config=sysgen:Constant_config
  logi_b22 : hdlBasic/Constant  const=-0.6451612903225806272544673447555396705865859985351562500  gui_display_data_type=Fixed-point  arith_type=Signed (2's comp)  n_bits=32  bin_pt=30  preci_type=Double  exp_width=8  frac_width=24  explicit_period=on  period=1  XmcBlockStatus=1  maskContainerNames=tabcontainer1  block_type=constant  block_config=sysgen:Constant_config
  logi_b23 : hdlBasic/Constant  const=-0.6290322580645161254508934689511079341173171997070312500  gui_display_data_type=Fixed-point  arith_type=Signed (2's comp)  n_bits=32  bin_pt=30  preci_type=Double  exp_width=8  frac_width=24  explicit_period=on  period=1  XmcBlockStatus=1  maskContainerNames=tabcontainer1  block_type=constant  block_config=sysgen:Constant_config
  logi_b24 : hdlBasic/Constant  const=-0.6129032258064516236473195931466761976480484008789062500  gui_display_data_type=Fixed-point  arith_type=Signed (2's comp)  n_bits=32  bin_pt=30  preci_type=Double  exp_width=8  frac_width=24  explicit_period=on  period=1  XmcBlockStatus=1  maskContainerNames=tabcontainer1  block_type=constant  block_config=sysgen:Constant_config
  logi_b25 : hdlBasic/Constant  const=-0.5967741935483871218437457173422444611787796020507812500  gui_display_data_type=Fixed-point  arith_type=Signed (2's comp)  n_bits=32  bin_pt=30  preci_type=Double  exp_width=8  frac_width=24  explicit_period=on  period=1  XmcBlockStatus=1  maskContainerNames=tabcontainer1  block_type=constant  block_config=sysgen:Constant_config
  logi_b26 : hdlBasic/Constant  const=-0.5806451612903225090178693790221586823463439941406250000  gui_display_data_type=Fixed-point  arith_type=Signed (2's comp)  n_bits=32  bin_pt=30  preci_type=Double  exp_width=8  frac_width=24  explicit_period=on  period=1  XmcBlockStatus=1  maskContainerNames=tabcontainer1  block_type=constant  block_config=sysgen:Constant_config
  logi_b27 : hdlBasic/Constant  const=-0.5645161290322580072142955032177269458770751953125000000  gui_display_data_type=Fixed-point  arith_type=Signed (2's comp)  n_bits=32  bin_pt=30  preci_type=Double  exp_width=8  frac_width=24  explicit_period=on  period=1  XmcBlockStatus=1  maskContainerNames=tabcontainer1  block_type=constant  block_config=sysgen:Constant_config
  logi_b28 : hdlBasic/Constant  const=-0.5483870967741935054107216274132952094078063964843750000  gui_display_data_type=Fixed-point  arith_type=Signed (2's comp)  n_bits=32  bin_pt=30  preci_type=Double  exp_width=8  frac_width=24  explicit_period=on  period=1  XmcBlockStatus=1  maskContainerNames=tabcontainer1  block_type=constant  block_config=sysgen:Constant_config
  logi_b29 : hdlBasic/Constant  const=-0.5322580645161290036071477516088634729385375976562500000  gui_display_data_type=Fixed-point  arith_type=Signed (2's comp)  n_bits=32  bin_pt=30  preci_type=Double  exp_width=8  frac_width=24  explicit_period=on  period=1  XmcBlockStatus=1  maskContainerNames=tabcontainer1  block_type=constant  block_config=sysgen:Constant_config
  logi_b3 : hdlBasic/Constant  const=-0.9516129032258063835669759100710507482290267944335937500  gui_display_data_type=Fixed-point  arith_type=Signed (2's comp)  n_bits=32  bin_pt=30  preci_type=Double  exp_width=8  frac_width=24  explicit_period=on  period=1  XmcBlockStatus=1  maskContainerNames=tabcontainer1  block_type=constant  block_config=sysgen:Constant_config
  logi_b30 : hdlBasic/Constant  const=-0.5161290322580645018035738758044317364692687988281250000  gui_display_data_type=Fixed-point  arith_type=Signed (2's comp)  n_bits=32  bin_pt=30  preci_type=Double  exp_width=8  frac_width=24  explicit_period=on  period=1  XmcBlockStatus=1  maskContainerNames=tabcontainer1  block_type=constant  block_config=sysgen:Constant_config
  logi_b31 : hdlBasic/Constant  const=-0.5000000000000000000000000000000000000000000000000000000  gui_display_data_type=Fixed-point  arith_type=Signed (2's comp)  n_bits=32  bin_pt=30  preci_type=Double  exp_width=8  frac_width=24  explicit_period=on  period=1  XmcBlockStatus=1  maskContainerNames=tabcontainer1  block_type=constant  block_config=sysgen:Constant_config
  logi_b32 : hdlBasic/Constant  const=-0.4838709677419354981964261241955682635307312011718750000  gui_display_data_type=Fixed-point  arith_type=Signed (2's comp)  n_bits=32  bin_pt=30  preci_type=Double  exp_width=8  frac_width=24  explicit_period=on  period=1  XmcBlockStatus=1  maskContainerNames=tabcontainer1  block_type=constant  block_config=sysgen:Constant_config
  logi_b33 : hdlBasic/Constant  const=-0.4677419354838709408817010171333095058798789978027343750  gui_display_data_type=Fixed-point  arith_type=Signed (2's comp)  n_bits=32  bin_pt=30  preci_type=Double  exp_width=8  frac_width=24  explicit_period=on  period=1  XmcBlockStatus=1  maskContainerNames=tabcontainer1  block_type=constant  block_config=sysgen:Constant_config
  logi_b34 : hdlBasic/Constant  const=-0.4516129032258064390781271413288777694106101989746093750  gui_display_data_type=Fixed-point  arith_type=Signed (2's comp)  n_bits=32  bin_pt=30  preci_type=Double  exp_width=8  frac_width=24  explicit_period=on  period=1  XmcBlockStatus=1  maskContainerNames=tabcontainer1  block_type=constant  block_config=sysgen:Constant_config
  logi_b35 : hdlBasic/Constant  const=-0.4354838709677419372745532655244460329413414001464843750  gui_display_data_type=Fixed-point  arith_type=Signed (2's comp)  n_bits=32  bin_pt=30  preci_type=Double  exp_width=8  frac_width=24  explicit_period=on  period=1  XmcBlockStatus=1  maskContainerNames=tabcontainer1  block_type=constant  block_config=sysgen:Constant_config
  logi_b36 : hdlBasic/Constant  const=-0.4193548387096773799598281584621872752904891967773437500  gui_display_data_type=Fixed-point  arith_type=Signed (2's comp)  n_bits=32  bin_pt=30  preci_type=Double  exp_width=8  frac_width=24  explicit_period=on  period=1  XmcBlockStatus=1  maskContainerNames=tabcontainer1  block_type=constant  block_config=sysgen:Constant_config
  logi_b37 : hdlBasic/Constant  const=-0.4032258064516128781562542826577555388212203979492187500  gui_display_data_type=Fixed-point  arith_type=Signed (2's comp)  n_bits=32  bin_pt=30  preci_type=Double  exp_width=8  frac_width=24  explicit_period=on  period=1  XmcBlockStatus=1  maskContainerNames=tabcontainer1  block_type=constant  block_config=sysgen:Constant_config
  logi_b38 : hdlBasic/Constant  const=-0.3870967741935483763526804068533238023519515991210937500  gui_display_data_type=Fixed-point  arith_type=Signed (2's comp)  n_bits=32  bin_pt=30  preci_type=Double  exp_width=8  frac_width=24  explicit_period=on  period=1  XmcBlockStatus=1  maskContainerNames=tabcontainer1  block_type=constant  block_config=sysgen:Constant_config
  logi_b39 : hdlBasic/Constant  const=-0.3709677419354838745491065310488920658826828002929687500  gui_display_data_type=Fixed-point  arith_type=Signed (2's comp)  n_bits=32  bin_pt=30  preci_type=Double  exp_width=8  frac_width=24  explicit_period=on  period=1  XmcBlockStatus=1  maskContainerNames=tabcontainer1  block_type=constant  block_config=sysgen:Constant_config
  logi_b4 : hdlBasic/Constant  const=-0.9354838709677418817634020342666190117597579956054687500  gui_display_data_type=Fixed-point  arith_type=Signed (2's comp)  n_bits=32  bin_pt=30  preci_type=Double  exp_width=8  frac_width=24  explicit_period=on  period=1  XmcBlockStatus=1  maskContainerNames=tabcontainer1  block_type=constant  block_config=sysgen:Constant_config
  logi_b40 : hdlBasic/Constant  const=-0.3548387096774193727455326552444603294134140014648437500  gui_display_data_type=Fixed-point  arith_type=Signed (2's comp)  n_bits=32  bin_pt=30  preci_type=Double  exp_width=8  frac_width=24  explicit_period=on  period=1  XmcBlockStatus=1  maskContainerNames=tabcontainer1  block_type=constant  block_config=sysgen:Constant_config
  logi_b41 : hdlBasic/Constant  const=-0.3387096774193548154308075481822015717625617980957031250  gui_display_data_type=Fixed-point  arith_type=Signed (2's comp)  n_bits=32  bin_pt=30  preci_type=Double  exp_width=8  frac_width=24  explicit_period=on  period=1  XmcBlockStatus=1  maskContainerNames=tabcontainer1  block_type=constant  block_config=sysgen:Constant_config
  logi_b42 : hdlBasic/Constant  const=-0.3225806451612903136272336723777698352932929992675781250  gui_display_data_type=Fixed-point  arith_type=Signed (2's comp)  n_bits=32  bin_pt=30  preci_type=Double  exp_width=8  frac_width=24  explicit_period=on  period=1  XmcBlockStatus=1  maskContainerNames=tabcontainer1  block_type=constant  block_config=sysgen:Constant_config
  logi_b43 : hdlBasic/Constant  const=-0.3064516129032258118236597965733380988240242004394531250  gui_display_data_type=Fixed-point  arith_type=Signed (2's comp)  n_bits=32  bin_pt=30  preci_type=Double  exp_width=8  frac_width=24  explicit_period=on  period=1  XmcBlockStatus=1  maskContainerNames=tabcontainer1  block_type=constant  block_config=sysgen:Constant_config
  logi_b44 : hdlBasic/Constant  const=-0.2903225806451612545089346895110793411731719970703125000  gui_display_data_type=Fixed-point  arith_type=Signed (2's comp)  n_bits=32  bin_pt=30  preci_type=Double  exp_width=8  frac_width=24  explicit_period=on  period=1  XmcBlockStatus=1  maskContainerNames=tabcontainer1  block_type=constant  block_config=sysgen:Constant_config
  logi_b45 : hdlBasic/Constant  const=-0.2741935483870967527053608137066476047039031982421875000  gui_display_data_type=Fixed-point  arith_type=Signed (2's comp)  n_bits=32  bin_pt=30  preci_type=Double  exp_width=8  frac_width=24  explicit_period=on  period=1  XmcBlockStatus=1  maskContainerNames=tabcontainer1  block_type=constant  block_config=sysgen:Constant_config
  logi_b46 : hdlBasic/Constant  const=-0.2580645161290322509017869379022158682346343994140625000  gui_display_data_type=Fixed-point  arith_type=Signed (2's comp)  n_bits=32  bin_pt=30  preci_type=Double  exp_width=8  frac_width=24  explicit_period=on  period=1  XmcBlockStatus=1  maskContainerNames=tabcontainer1  block_type=constant  block_config=sysgen:Constant_config
  logi_b47 : hdlBasic/Constant  const=-0.2419354838709677490982130620977841317653656005859375000  gui_display_data_type=Fixed-point  arith_type=Signed (2's comp)  n_bits=32  bin_pt=30  preci_type=Double  exp_width=8  frac_width=24  explicit_period=on  period=1  XmcBlockStatus=1  maskContainerNames=tabcontainer1  block_type=constant  block_config=sysgen:Constant_config
  logi_b48 : hdlBasic/Constant  const=-0.2258064516129032195390635706644388847053050994873046875  gui_display_data_type=Fixed-point  arith_type=Signed (2's comp)  n_bits=32  bin_pt=30  preci_type=Double  exp_width=8  frac_width=24  explicit_period=on  period=1  XmcBlockStatus=1  maskContainerNames=tabcontainer1  block_type=constant  block_config=sysgen:Constant_config
  logi_b49 : hdlBasic/Constant  const=-0.2096774193548386899799140792310936376452445983886718750  gui_display_data_type=Fixed-point  arith_type=Signed (2's comp)  n_bits=32  bin_pt=30  preci_type=Double  exp_width=8  frac_width=24  explicit_period=on  period=1  XmcBlockStatus=1  maskContainerNames=tabcontainer1  block_type=constant  block_config=sysgen:Constant_config
  logi_b5 : hdlBasic/Constant  const=-0.9193548387096773799598281584621872752904891967773437500  gui_display_data_type=Fixed-point  arith_type=Signed (2's comp)  n_bits=32  bin_pt=30  preci_type=Double  exp_width=8  frac_width=24  explicit_period=on  period=1  XmcBlockStatus=1  maskContainerNames=tabcontainer1  block_type=constant  block_config=sysgen:Constant_config
  logi_b50 : hdlBasic/Constant  const=-0.1935483870967741881763402034266619011759757995605468750  gui_display_data_type=Fixed-point  arith_type=Signed (2's comp)  n_bits=32  bin_pt=30  preci_type=Double  exp_width=8  frac_width=24  explicit_period=on  period=1  XmcBlockStatus=1  maskContainerNames=tabcontainer1  block_type=constant  block_config=sysgen:Constant_config
  logi_b51 : hdlBasic/Constant  const=-0.1774193548387096863727663276222301647067070007324218750  gui_display_data_type=Fixed-point  arith_type=Signed (2's comp)  n_bits=32  bin_pt=30  preci_type=Double  exp_width=8  frac_width=24  explicit_period=on  period=1  XmcBlockStatus=1  maskContainerNames=tabcontainer1  block_type=constant  block_config=sysgen:Constant_config
  logi_b52 : hdlBasic/Constant  const=-0.1612903225806451568136168361888849176466464996337890625  gui_display_data_type=Fixed-point  arith_type=Signed (2's comp)  n_bits=32  bin_pt=30  preci_type=Double  exp_width=8  frac_width=24  explicit_period=on  period=1  XmcBlockStatus=1  maskContainerNames=tabcontainer1  block_type=constant  block_config=sysgen:Constant_config
  logi_b53 : hdlBasic/Constant  const=-0.1451612903225806272544673447555396705865859985351562500  gui_display_data_type=Fixed-point  arith_type=Signed (2's comp)  n_bits=32  bin_pt=30  preci_type=Double  exp_width=8  frac_width=24  explicit_period=on  period=1  XmcBlockStatus=1  maskContainerNames=tabcontainer1  block_type=constant  block_config=sysgen:Constant_config
  logi_b54 : hdlBasic/Constant  const=-0.1290322580645161254508934689511079341173171997070312500  gui_display_data_type=Fixed-point  arith_type=Signed (2's comp)  n_bits=32  bin_pt=30  preci_type=Double  exp_width=8  frac_width=24  explicit_period=on  period=1  XmcBlockStatus=1  maskContainerNames=tabcontainer1  block_type=constant  block_config=sysgen:Constant_config
  logi_b55 : hdlBasic/Constant  const=-0.1129032258064516097695317853322194423526525497436523438  gui_display_data_type=Fixed-point  arith_type=Signed (2's comp)  n_bits=32  bin_pt=30  preci_type=Double  exp_width=8  frac_width=24  explicit_period=on  period=1  XmcBlockStatus=1  maskContainerNames=tabcontainer1  block_type=constant  block_config=sysgen:Constant_config
  logi_b56 : hdlBasic/Constant  const=-0.0967741935483870940881701017133309505879878997802734375  gui_display_data_type=Fixed-point  arith_type=Signed (2's comp)  n_bits=32  bin_pt=30  preci_type=Double  exp_width=8  frac_width=24  explicit_period=on  period=1  XmcBlockStatus=1  maskContainerNames=tabcontainer1  block_type=constant  block_config=sysgen:Constant_config
  logi_b57 : hdlBasic/Constant  const=-0.0806451612903225784068084180944424588233232498168945312  gui_display_data_type=Fixed-point  arith_type=Signed (2's comp)  n_bits=32  bin_pt=30  preci_type=Double  exp_width=8  frac_width=24  explicit_period=on  period=1  XmcBlockStatus=1  maskContainerNames=tabcontainer1  block_type=constant  block_config=sysgen:Constant_config
  logi_b58 : hdlBasic/Constant  const=-0.0645161290322580627254467344755539670586585998535156250  gui_display_data_type=Fixed-point  arith_type=Signed (2's comp)  n_bits=32  bin_pt=30  preci_type=Double  exp_width=8  frac_width=24  explicit_period=on  period=1  XmcBlockStatus=1  maskContainerNames=tabcontainer1  block_type=constant  block_config=sysgen:Constant_config
  logi_b59 : hdlBasic/Constant  const=-0.0483870967741935470440850508566654752939939498901367188  gui_display_data_type=Fixed-point  arith_type=Signed (2's comp)  n_bits=32  bin_pt=30  preci_type=Double  exp_width=8  frac_width=24  explicit_period=on  period=1  XmcBlockStatus=1  maskContainerNames=tabcontainer1  block_type=constant  block_config=sysgen:Constant_config
  logi_b6 : hdlBasic/Constant  const=-0.9032258064516128781562542826577555388212203979492187500  gui_display_data_type=Fixed-point  arith_type=Signed (2's comp)  n_bits=32  bin_pt=30  preci_type=Double  exp_width=8  frac_width=24  explicit_period=on  period=1  XmcBlockStatus=1  maskContainerNames=tabcontainer1  block_type=constant  block_config=sysgen:Constant_config
  logi_b60 : hdlBasic/Constant  const=-0.0322580645161290313627233672377769835293292999267578125  gui_display_data_type=Fixed-point  arith_type=Signed (2's comp)  n_bits=32  bin_pt=30  preci_type=Double  exp_width=8  frac_width=24  explicit_period=on  period=1  XmcBlockStatus=1  maskContainerNames=tabcontainer1  block_type=constant  block_config=sysgen:Constant_config
  logi_b61 : hdlBasic/Constant  const=-0.0161290322580645156813616836188884917646646499633789062  gui_display_data_type=Fixed-point  arith_type=Signed (2's comp)  n_bits=32  bin_pt=30  preci_type=Double  exp_width=8  frac_width=24  explicit_period=on  period=1  XmcBlockStatus=1  maskContainerNames=tabcontainer1  block_type=constant  block_config=sysgen:Constant_config
  logi_b62 : hdlBasic/Constant  const=0.0000000000000000000000000000000000000000000000000000000  gui_display_data_type=Fixed-point  arith_type=Signed (2's comp)  n_bits=32  bin_pt=30  preci_type=Double  exp_width=8  frac_width=24  explicit_period=on  period=1  XmcBlockStatus=1  maskContainerNames=tabcontainer1  block_type=constant  block_config=sysgen:Constant_config
  logi_b63 : hdlBasic/Constant  const=0.0161290322580645156813616836188884917646646499633789062  gui_display_data_type=Fixed-point  arith_type=Signed (2's comp)  n_bits=32  bin_pt=30  preci_type=Double  exp_width=8  frac_width=24  explicit_period=on  period=1  XmcBlockStatus=1  maskContainerNames=tabcontainer1  block_type=constant  block_config=sysgen:Constant_config
  logi_b64 : hdlBasic/Constant  const=0.0322580645161290313627233672377769835293292999267578125  gui_display_data_type=Fixed-point  arith_type=Signed (2's comp)  n_bits=32  bin_pt=30  preci_type=Double  exp_width=8  frac_width=24  explicit_period=on  period=1  XmcBlockStatus=1  maskContainerNames=tabcontainer1  block_type=constant  block_config=sysgen:Constant_config
  logi_b65 : hdlBasic/Constant  const=0.0483870967741935470440850508566654752939939498901367188  gui_display_data_type=Fixed-point  arith_type=Signed (2's comp)  n_bits=32  bin_pt=30  preci_type=Double  exp_width=8  frac_width=24  explicit_period=on  period=1  XmcBlockStatus=1  maskContainerNames=tabcontainer1  block_type=constant  block_config=sysgen:Constant_config
  logi_b66 : hdlBasic/Constant  const=0.0645161290322580627254467344755539670586585998535156250  gui_display_data_type=Fixed-point  arith_type=Signed (2's comp)  n_bits=32  bin_pt=30  preci_type=Double  exp_width=8  frac_width=24  explicit_period=on  period=1  XmcBlockStatus=1  maskContainerNames=tabcontainer1  block_type=constant  block_config=sysgen:Constant_config
  logi_b67 : hdlBasic/Constant  const=0.0806451612903225784068084180944424588233232498168945312  gui_display_data_type=Fixed-point  arith_type=Signed (2's comp)  n_bits=32  bin_pt=30  preci_type=Double  exp_width=8  frac_width=24  explicit_period=on  period=1  XmcBlockStatus=1  maskContainerNames=tabcontainer1  block_type=constant  block_config=sysgen:Constant_config
  logi_b68 : hdlBasic/Constant  const=0.0967741935483870940881701017133309505879878997802734375  gui_display_data_type=Fixed-point  arith_type=Signed (2's comp)  n_bits=32  bin_pt=30  preci_type=Double  exp_width=8  frac_width=24  explicit_period=on  period=1  XmcBlockStatus=1  maskContainerNames=tabcontainer1  block_type=constant  block_config=sysgen:Constant_config
  logi_b69 : hdlBasic/Constant  const=0.1129032258064516097695317853322194423526525497436523438  gui_display_data_type=Fixed-point  arith_type=Signed (2's comp)  n_bits=32  bin_pt=30  preci_type=Double  exp_width=8  frac_width=24  explicit_period=on  period=1  XmcBlockStatus=1  maskContainerNames=tabcontainer1  block_type=constant  block_config=sysgen:Constant_config
  logi_b7 : hdlBasic/Constant  const=-0.8870967741935483763526804068533238023519515991210937500  gui_display_data_type=Fixed-point  arith_type=Signed (2's comp)  n_bits=32  bin_pt=30  preci_type=Double  exp_width=8  frac_width=24  explicit_period=on  period=1  XmcBlockStatus=1  maskContainerNames=tabcontainer1  block_type=constant  block_config=sysgen:Constant_config
  logi_b70 : hdlBasic/Constant  const=0.1290322580645161254508934689511079341173171997070312500  gui_display_data_type=Fixed-point  arith_type=Signed (2's comp)  n_bits=32  bin_pt=30  preci_type=Double  exp_width=8  frac_width=24  explicit_period=on  period=1  XmcBlockStatus=1  maskContainerNames=tabcontainer1  block_type=constant  block_config=sysgen:Constant_config
  logi_b71 : hdlBasic/Constant  const=0.1451612903225806272544673447555396705865859985351562500  gui_display_data_type=Fixed-point  arith_type=Signed (2's comp)  n_bits=32  bin_pt=30  preci_type=Double  exp_width=8  frac_width=24  explicit_period=on  period=1  XmcBlockStatus=1  maskContainerNames=tabcontainer1  block_type=constant  block_config=sysgen:Constant_config
  logi_b72 : hdlBasic/Constant  const=0.1612903225806451568136168361888849176466464996337890625  gui_display_data_type=Fixed-point  arith_type=Signed (2's comp)  n_bits=32  bin_pt=30  preci_type=Double  exp_width=8  frac_width=24  explicit_period=on  period=1  XmcBlockStatus=1  maskContainerNames=tabcontainer1  block_type=constant  block_config=sysgen:Constant_config
  logi_b73 : hdlBasic/Constant  const=0.1774193548387096863727663276222301647067070007324218750  gui_display_data_type=Fixed-point  arith_type=Signed (2's comp)  n_bits=32  bin_pt=30  preci_type=Double  exp_width=8  frac_width=24  explicit_period=on  period=1  XmcBlockStatus=1  maskContainerNames=tabcontainer1  block_type=constant  block_config=sysgen:Constant_config
  logi_b74 : hdlBasic/Constant  const=0.1935483870967741881763402034266619011759757995605468750  gui_display_data_type=Fixed-point  arith_type=Signed (2's comp)  n_bits=32  bin_pt=30  preci_type=Double  exp_width=8  frac_width=24  explicit_period=on  period=1  XmcBlockStatus=1  maskContainerNames=tabcontainer1  block_type=constant  block_config=sysgen:Constant_config
  logi_b75 : hdlBasic/Constant  const=0.2096774193548386899799140792310936376452445983886718750  gui_display_data_type=Fixed-point  arith_type=Signed (2's comp)  n_bits=32  bin_pt=30  preci_type=Double  exp_width=8  frac_width=24  explicit_period=on  period=1  XmcBlockStatus=1  maskContainerNames=tabcontainer1  block_type=constant  block_config=sysgen:Constant_config
  logi_b76 : hdlBasic/Constant  const=0.2258064516129032195390635706644388847053050994873046875  gui_display_data_type=Fixed-point  arith_type=Signed (2's comp)  n_bits=32  bin_pt=30  preci_type=Double  exp_width=8  frac_width=24  explicit_period=on  period=1  XmcBlockStatus=1  maskContainerNames=tabcontainer1  block_type=constant  block_config=sysgen:Constant_config
  logi_b77 : hdlBasic/Constant  const=0.2419354838709677490982130620977841317653656005859375000  gui_display_data_type=Fixed-point  arith_type=Signed (2's comp)  n_bits=32  bin_pt=30  preci_type=Double  exp_width=8  frac_width=24  explicit_period=on  period=1  XmcBlockStatus=1  maskContainerNames=tabcontainer1  block_type=constant  block_config=sysgen:Constant_config
  logi_b78 : hdlBasic/Constant  const=0.2580645161290322509017869379022158682346343994140625000  gui_display_data_type=Fixed-point  arith_type=Signed (2's comp)  n_bits=32  bin_pt=30  preci_type=Double  exp_width=8  frac_width=24  explicit_period=on  period=1  XmcBlockStatus=1  maskContainerNames=tabcontainer1  block_type=constant  block_config=sysgen:Constant_config
  logi_b79 : hdlBasic/Constant  const=0.2741935483870967527053608137066476047039031982421875000  gui_display_data_type=Fixed-point  arith_type=Signed (2's comp)  n_bits=32  bin_pt=30  preci_type=Double  exp_width=8  frac_width=24  explicit_period=on  period=1  XmcBlockStatus=1  maskContainerNames=tabcontainer1  block_type=constant  block_config=sysgen:Constant_config
  logi_b8 : hdlBasic/Constant  const=-0.8709677419354838745491065310488920658826828002929687500  gui_display_data_type=Fixed-point  arith_type=Signed (2's comp)  n_bits=32  bin_pt=30  preci_type=Double  exp_width=8  frac_width=24  explicit_period=on  period=1  XmcBlockStatus=1  maskContainerNames=tabcontainer1  block_type=constant  block_config=sysgen:Constant_config
  logi_b80 : hdlBasic/Constant  const=0.2903225806451612545089346895110793411731719970703125000  gui_display_data_type=Fixed-point  arith_type=Signed (2's comp)  n_bits=32  bin_pt=30  preci_type=Double  exp_width=8  frac_width=24  explicit_period=on  period=1  XmcBlockStatus=1  maskContainerNames=tabcontainer1  block_type=constant  block_config=sysgen:Constant_config
  logi_b81 : hdlBasic/Constant  const=0.3064516129032258118236597965733380988240242004394531250  gui_display_data_type=Fixed-point  arith_type=Signed (2's comp)  n_bits=32  bin_pt=30  preci_type=Double  exp_width=8  frac_width=24  explicit_period=on  period=1  XmcBlockStatus=1  maskContainerNames=tabcontainer1  block_type=constant  block_config=sysgen:Constant_config
  logi_b82 : hdlBasic/Constant  const=0.3225806451612903136272336723777698352932929992675781250  gui_display_data_type=Fixed-point  arith_type=Signed (2's comp)  n_bits=32  bin_pt=30  preci_type=Double  exp_width=8  frac_width=24  explicit_period=on  period=1  XmcBlockStatus=1  maskContainerNames=tabcontainer1  block_type=constant  block_config=sysgen:Constant_config
  logi_b83 : hdlBasic/Constant  const=0.3387096774193548154308075481822015717625617980957031250  gui_display_data_type=Fixed-point  arith_type=Signed (2's comp)  n_bits=32  bin_pt=30  preci_type=Double  exp_width=8  frac_width=24  explicit_period=on  period=1  XmcBlockStatus=1  maskContainerNames=tabcontainer1  block_type=constant  block_config=sysgen:Constant_config
  logi_b84 : hdlBasic/Constant  const=0.3548387096774193727455326552444603294134140014648437500  gui_display_data_type=Fixed-point  arith_type=Signed (2's comp)  n_bits=32  bin_pt=30  preci_type=Double  exp_width=8  frac_width=24  explicit_period=on  period=1  XmcBlockStatus=1  maskContainerNames=tabcontainer1  block_type=constant  block_config=sysgen:Constant_config
  logi_b85 : hdlBasic/Constant  const=0.3709677419354838745491065310488920658826828002929687500  gui_display_data_type=Fixed-point  arith_type=Signed (2's comp)  n_bits=32  bin_pt=30  preci_type=Double  exp_width=8  frac_width=24  explicit_period=on  period=1  XmcBlockStatus=1  maskContainerNames=tabcontainer1  block_type=constant  block_config=sysgen:Constant_config
  logi_b86 : hdlBasic/Constant  const=0.3870967741935483763526804068533238023519515991210937500  gui_display_data_type=Fixed-point  arith_type=Signed (2's comp)  n_bits=32  bin_pt=30  preci_type=Double  exp_width=8  frac_width=24  explicit_period=on  period=1  XmcBlockStatus=1  maskContainerNames=tabcontainer1  block_type=constant  block_config=sysgen:Constant_config
  logi_b87 : hdlBasic/Constant  const=0.4032258064516128781562542826577555388212203979492187500  gui_display_data_type=Fixed-point  arith_type=Signed (2's comp)  n_bits=32  bin_pt=30  preci_type=Double  exp_width=8  frac_width=24  explicit_period=on  period=1  XmcBlockStatus=1  maskContainerNames=tabcontainer1  block_type=constant  block_config=sysgen:Constant_config
  logi_b88 : hdlBasic/Constant  const=0.4193548387096773799598281584621872752904891967773437500  gui_display_data_type=Fixed-point  arith_type=Signed (2's comp)  n_bits=32  bin_pt=30  preci_type=Double  exp_width=8  frac_width=24  explicit_period=on  period=1  XmcBlockStatus=1  maskContainerNames=tabcontainer1  block_type=constant  block_config=sysgen:Constant_config
  logi_b89 : hdlBasic/Constant  const=0.4354838709677419372745532655244460329413414001464843750  gui_display_data_type=Fixed-point  arith_type=Signed (2's comp)  n_bits=32  bin_pt=30  preci_type=Double  exp_width=8  frac_width=24  explicit_period=on  period=1  XmcBlockStatus=1  maskContainerNames=tabcontainer1  block_type=constant  block_config=sysgen:Constant_config
  logi_b9 : hdlBasic/Constant  const=-0.8548387096774193727455326552444603294134140014648437500  gui_display_data_type=Fixed-point  arith_type=Signed (2's comp)  n_bits=32  bin_pt=30  preci_type=Double  exp_width=8  frac_width=24  explicit_period=on  period=1  XmcBlockStatus=1  maskContainerNames=tabcontainer1  block_type=constant  block_config=sysgen:Constant_config
  logi_b90 : hdlBasic/Constant  const=0.4516129032258064390781271413288777694106101989746093750  gui_display_data_type=Fixed-point  arith_type=Signed (2's comp)  n_bits=32  bin_pt=30  preci_type=Double  exp_width=8  frac_width=24  explicit_period=on  period=1  XmcBlockStatus=1  maskContainerNames=tabcontainer1  block_type=constant  block_config=sysgen:Constant_config
  logi_b91 : hdlBasic/Constant  const=0.4677419354838709408817010171333095058798789978027343750  gui_display_data_type=Fixed-point  arith_type=Signed (2's comp)  n_bits=32  bin_pt=30  preci_type=Double  exp_width=8  frac_width=24  explicit_period=on  period=1  XmcBlockStatus=1  maskContainerNames=tabcontainer1  block_type=constant  block_config=sysgen:Constant_config
  logi_b92 : hdlBasic/Constant  const=0.4838709677419354981964261241955682635307312011718750000  gui_display_data_type=Fixed-point  arith_type=Signed (2's comp)  n_bits=32  bin_pt=30  preci_type=Double  exp_width=8  frac_width=24  explicit_period=on  period=1  XmcBlockStatus=1  maskContainerNames=tabcontainer1  block_type=constant  block_config=sysgen:Constant_config
  logi_b93 : hdlBasic/Constant  const=0.5000000000000000000000000000000000000000000000000000000  gui_display_data_type=Fixed-point  arith_type=Signed (2's comp)  n_bits=32  bin_pt=30  preci_type=Double  exp_width=8  frac_width=24  explicit_period=on  period=1  XmcBlockStatus=1  maskContainerNames=tabcontainer1  block_type=constant  block_config=sysgen:Constant_config
  logi_b94 : hdlBasic/Constant  const=0.5161290322580645018035738758044317364692687988281250000  gui_display_data_type=Fixed-point  arith_type=Signed (2's comp)  n_bits=32  bin_pt=30  preci_type=Double  exp_width=8  frac_width=24  explicit_period=on  period=1  XmcBlockStatus=1  maskContainerNames=tabcontainer1  block_type=constant  block_config=sysgen:Constant_config
  logi_b95 : hdlBasic/Constant  const=0.5322580645161290036071477516088634729385375976562500000  gui_display_data_type=Fixed-point  arith_type=Signed (2's comp)  n_bits=32  bin_pt=30  preci_type=Double  exp_width=8  frac_width=24  explicit_period=on  period=1  XmcBlockStatus=1  maskContainerNames=tabcontainer1  block_type=constant  block_config=sysgen:Constant_config
  logi_b96 : hdlBasic/Constant  const=0.5483870967741935054107216274132952094078063964843750000  gui_display_data_type=Fixed-point  arith_type=Signed (2's comp)  n_bits=32  bin_pt=30  preci_type=Double  exp_width=8  frac_width=24  explicit_period=on  period=1  XmcBlockStatus=1  maskContainerNames=tabcontainer1  block_type=constant  block_config=sysgen:Constant_config
  logi_b97 : hdlBasic/Constant  const=0.5645161290322580072142955032177269458770751953125000000  gui_display_data_type=Fixed-point  arith_type=Signed (2's comp)  n_bits=32  bin_pt=30  preci_type=Double  exp_width=8  frac_width=24  explicit_period=on  period=1  XmcBlockStatus=1  maskContainerNames=tabcontainer1  block_type=constant  block_config=sysgen:Constant_config
  logi_b98 : hdlBasic/Constant  const=0.5806451612903225090178693790221586823463439941406250000  gui_display_data_type=Fixed-point  arith_type=Signed (2's comp)  n_bits=32  bin_pt=30  preci_type=Double  exp_width=8  frac_width=24  explicit_period=on  period=1  XmcBlockStatus=1  maskContainerNames=tabcontainer1  block_type=constant  block_config=sysgen:Constant_config
  logi_b99 : hdlBasic/Constant  const=0.5967741935483871218437457173422444611787796020507812500  gui_display_data_type=Fixed-point  arith_type=Signed (2's comp)  n_bits=32  bin_pt=30  preci_type=Double  exp_width=8  frac_width=24  explicit_period=on  period=1  XmcBlockStatus=1  maskContainerNames=tabcontainer1  block_type=constant  block_config=sysgen:Constant_config
  logical_x0 : hdlBasic/Mux  inputs=2  en=off  latency=0  precision=Full  arith_type=Unsigned  n_bits=16  bin_pt=14  quantization=Truncate  overflow=Wrap  XmcBlockStatus=1  maskContainerNames=tabcontainer1  block_type=mux  block_config=sysgen:Mux_config
  logical_y0 : hdlBasic/Mux  inputs=2  en=off  latency=0  precision=Full  arith_type=Unsigned  n_bits=16  bin_pt=14  quantization=Truncate  overflow=Wrap  XmcBlockStatus=1  maskContainerNames=tabcontainer1  block_type=mux  block_config=sysgen:Mux_config
  mux{1..112} (112 alike) : hdlBasic/Mux  inputs=2  en=off  latency=1  precision=Full  arith_type=Unsigned  n_bits=16  bin_pt=14  quantization=Truncate  overflow=Wrap  XmcBlockStatus=1  maskContainerNames=tabcontainer1  block_type=mux  block_config=sysgen:Mux_config
  rela{1..112} (112 alike) : hdlBasic/Relational  mode=a>=b  op_type=Bool  en=off  latency=1  XmcBlockStatus=1  maskContainerNames=tabcontainer1  block_type=relational  block_config=sysgen:Relational_config
  Output : Outport
  wires:
  addsub9/1 -> mux11/3
  In4/1 -> Gate_In2/1
  addsub13/1 -> mux15/3
  In3/1 -> Gate_In1/1
  addsub1/1 -> mux3/3
  addsub5/1 -> mux7/3
  addsub3/1 -> mux5/3
  rela1/1 -> mux1/1
  addsub7/1 -> mux9/3
  addsub11/1 -> mux13/3
  addsub15/1 -> mux17/3
  bool1/1 -> logical_x0/1, logical_y0/1
  Constant3/1 -> AddSub19/2
  Constant/1 -> AddSub18/2
  AddSub19/1 -> Mult/2
  AddSub18/1 -> Negate/1
  Constant4/1 -> Mult1/2
  AddSub22/1 -> Slice3/1
  AddSub21/1 -> AddSub22/1
  AddSub20/1 -> AddSub21/1
  Mult1/1 -> AddSub20/1
  Negate/1 -> AddSub19/1
  Mult/1 -> Slice2/1
  Gate_In2/1 -> bool1/2, logical_x0/2, logical_y0/3
  Gate_In1/1 -> bool1/1, logical_x0/3, logical_y0/2
  rela3/1 -> mux3/1
  mux1/1 -> mux3/2, addsub1/1
  rela5/1 -> mux5/1
  mux3/1 -> mux5/2, addsub3/1
  rela7/1 -> mux7/1
  mux5/1 -> mux7/2, addsub5/1
  rela9/1 -> mux9/1
  mux7/1 -> mux9/2, addsub7/1
  rela11/1 -> mux11/1
  mux9/1 -> mux11/2, addsub9/1
  rela13/1 -> mux13/1
  mux11/1 -> mux13/2, addsub11/1
  rela15/1 -> mux15/1
  mux13/1 -> mux15/2, addsub13/1
  rela17/1 -> mux17/1
  mux15/1 -> mux17/2, addsub15/1
  mux4/1 -> mux6/2, addsub4/1
  mux14/1 -> mux16/2, addsub14/1
  rela18/1 -> mux18/1
  rela10/1 -> mux10/1
  logi_b3/1 -> rela8/2, rela7/2
  addsub4/1 -> mux6/3
  addsub12/1 -> mux14/3
  rela12/1 -> mux12/1
  logi_b1/1 -> rela4/2, rela3/2
  rela2/1 -> mux2/1
  addsub6/1 -> mux8/3
  mux6/1 -> mux8/2, addsub6/1
  rela14/1 -> mux14/1
  logi_b4/1 -> rela10/2, rela9/2
  mux8/1 -> mux10/2, addsub8/1
  logi_b7/1 -> rela16/2, rela15/2
  rela16/1 -> mux16/1
  logi_b0/1 -> rela2/2, rela1/2
  mux16/1 -> mux18/2, addsub16/1
  logi_b5/1 -> rela12/2, rela11/2
  mux2/1 -> mux4/2, addsub2/1
  rela8/1 -> mux8/1
  mux12/1 -> mux14/2, addsub12/1
  rela6/1 -> mux6/1
  logi_b2/1 -> rela5/2, rela6/2
  addsub8/1 -> mux10/3
  addsub14/1 -> mux16/3
  mux10/1 -> mux12/2, addsub10/1
  logi_b6/1 -> rela14/2, rela13/2
  rela4/1 -> mux4/1
  addsub10/1 -> mux12/3
  addsub16/1 -> mux18/3
  logi_b8/1 -> rela18/2, rela17/2
  addsub2/1 -> mux4/3
  Constant6/1 -> mux2/2
  Constant1/1 -> mux1/2
  Delay59/1 -> Mult1/1
  Delay60/1 -> Mult/1
  Delay61/1 -> AddSub21/2
  rela36/1 -> mux36/1
  rela32/1 -> mux32/1
  mux29/1 -> mux31/2, addsub29/1
  rela28/1 -> mux28/1
  rela30/1 -> mux30/1
  mux28/1 -> mux30/2, addsub28/1
  addsub28/1 -> mux30/3
  rela24/1 -> mux24/1
  mux24/1 -> mux26/2, addsub24/1
  addsub19/1 -> mux21/3
  addsub25/1 -> mux27/3
  logi_b11/1 -> rela24/2, rela23/2
  rela35/1 -> mux35/1
  rela29/1 -> mux29/1
  addsub32/1 -> mux34/3
  rela34/1 -> mux34/1
  rela27/1 -> mux27/1
  logi_b13/1 -> rela28/2, rela27/2
  logi_b15/1 -> rela32/2, rela31/2
  rela26/1 -> mux26/1
  addsub22/1 -> mux24/3
  logi_b17/1 -> rela36/2, rela35/2
  addsub29/1 -> mux31/3
  mux26/1 -> mux28/2, addsub26/1
  addsub26/1 -> mux28/3
  rela23/1 -> mux23/1
  rela33/1 -> mux33/1
  mux32/1 -> mux34/2, addsub32/1
  addsub33/1 -> mux35/3
  mux27/1 -> mux29/2, addsub27/1
  addsub27/1 -> mux29/3
  addsub24/1 -> mux26/3
  mux30/1 -> mux32/2, addsub30/1
  logi_b12/1 -> rela26/2, rela25/2
  rela22/1 -> mux22/1
  rela31/1 -> mux31/1
  mux33/1 -> mux35/2, addsub33/1
  logi_b10/1 -> rela22/2, rela21/2
  logi_b16/1 -> rela34/2, rela33/2
  addsub20/1 -> mux22/3
  addsub34/1 -> mux36/3
  mux25/1 -> mux27/2, addsub25/1
  addsub23/1 -> mux25/3
  mux19/1 -> mux21/2, addsub19/1
  addsub21/1 -> mux23/3
  mux34/1 -> mux36/2, addsub34/1
  mux20/1 -> mux22/2, addsub20/1
  mux23/1 -> mux25/2, addsub23/1
  mux21/1 -> mux23/2, addsub21/1
  addsub30/1 -> mux32/3
  addsub31/1 -> mux33/3
  logi_b14/1 -> rela30/2, rela29/2
  rela21/1 -> mux21/1
  mux22/1 -> mux24/2, addsub22/1
  mux31/1 -> mux33/2, addsub31/1
  rela25/1 -> mux25/1
  mux97/1 -> mux99/2, addsub97/1
  logi_b49/1 -> rela100/2, rela99/2
  rela99/1 -> mux99/1
  addsub98/1 -> mux100/3
  rela100/1 -> mux100/1
  addsub97/1 -> mux99/3
  mux98/1 -> mux100/2, addsub98/1
  addsub18/1 -> mux20/3
  addsub17/1 -> mux19/3
  rela19/1 -> mux19/1
  mux18/1 -> mux20/2, addsub18/1
  mux17/1 -> mux19/2, addsub17/1
  rela20/1 -> mux20/1
  logi_b9/1 -> rela20/2, rela19/2
  addsub36/1 -> mux38/3
  addsub35/1 -> mux37/3
  rela37/1 -> mux37/1
  mux36/1 -> mux38/2, addsub36/1
  mux35/1 -> mux37/2, addsub35/1
  rela38/1 -> mux38/1
  logi_b18/1 -> rela38/2, rela37/2
  mux49/1 -> mux51/2, addsub49/1
  addsub48/1 -> mux50/3
  mux38/1 -> mux40/2, addsub38/1
  addsub49/1 -> mux51/3
  mux52/1 -> mux54/2, addsub52/1
  rela43/1 -> mux43/1
  mux43/1 -> mux45/2, addsub43/1
  addsub52/1 -> mux54/3
  logi_b25/1 -> rela52/2, rela51/2
  rela50/1 -> mux50/1
  mux39/1 -> mux41/2, addsub39/1
  logi_b26/1 -> rela54/2, rela53/2
  addsub40/1 -> mux42/3
  rela48/1 -> mux48/1
  mux53/1 -> mux55/2, addsub53/1
  mux44/1 -> mux46/2, addsub44/1
  rela52/1 -> mux52/1
  addsub54/1 -> mux56/3
  logi_b22/1 -> rela46/2, rela45/2
  addsub53/1 -> mux55/3
  rela54/1 -> mux54/1
  mux54/1 -> mux56/2, addsub54/1
  addsub50/1 -> mux52/3
  rela39/1 -> mux39/1
  mux37/1 -> mux39/2, addsub37/1
  addsub47/1 -> mux49/3
  mux42/1 -> mux44/2, addsub42/1
  logi_b23/1 -> rela48/2, rela47/2
  rela45/1 -> mux45/1
  logi_b24/1 -> rela50/2, rela49/2
  addsub44/1 -> mux46/3
  mux46/1 -> mux48/2, addsub46/1
  addsub39/1 -> mux41/3
  rela55/1 -> mux55/1
  addsub43/1 -> mux45/3
  addsub41/1 -> mux43/3
  rela47/1 -> mux47/1
  addsub38/1 -> mux40/3
  logi_b19/1 -> rela40/2, rela39/2
  addsub37/1 -> mux39/3
  rela42/1 -> mux42/1
  logi_b27/1 -> rela56/2, rela55/2
  mux41/1 -> mux43/2, addsub41/1
  logi_b21/1 -> rela44/2, rela43/2
  rela44/1 -> mux44/1
  addsub42/1 -> mux44/3
  mux51/1 -> mux53/2, addsub51/1
  rela51/1 -> mux51/1
  rela53/1 -> mux53/1
  addsub46/1 -> mux48/3
  mux47/1 -> mux49/2, addsub47/1
  rela46/1 -> mux46/1
  mux48/1 -> mux50/2, addsub48/1
  rela40/1 -> mux40/1
  logi_b20/1 -> rela42/2, rela41/2
  rela49/1 -> mux49/1
  rela41/1 -> mux41/1
  mux50/1 -> mux52/2, addsub50/1
  addsub51/1 -> mux53/3
  mux45/1 -> mux47/2, addsub45/1
  addsub45/1 -> mux47/3
  rela56/1 -> mux56/1
  mux40/1 -> mux42/2, addsub40/1
  addsub59/1 -> mux61/3
  addsub63/1 -> mux65/3
  addsub74/1 -> mux76/3
  addsub96/1 -> mux98/3
  logi_b45/1 -> rela92/2, rela91/2
  rela79/1 -> mux79/1
  rela97/1 -> mux97/1
  mux90/1 -> mux92/2, addsub90/1
  rela60/1 -> mux60/1
  addsub69/1 -> mux71/3
  rela91/1 -> mux91/1
  addsub95/1 -> mux97/3
  addsub62/1 -> mux64/3
  rela96/1 -> mux96/1
  mux96/1 -> mux98/2, addsub96/1
  addsub80/1 -> mux82/3
  addsub93/1 -> mux95/3
  logi_b47/1 -> rela96/2, rela95/2
  logi_b48/1 -> rela98/2, rela97/2
  rela59/1 -> mux59/1
  addsub91/1 -> mux93/3
  mux93/1 -> mux95/2, addsub93/1
  addsub70/1 -> mux72/3
  addsub66/1 -> mux68/3
  rela68/1 -> mux68/1
  rela94/1 -> mux94/1
  rela86/1 -> mux86/1
  logi_b30/1 -> rela62/2, rela61/2
  addsub89/1 -> mux91/3
  addsub57/1 -> mux59/3
  mux94/1 -> mux96/2, addsub94/1
  mux92/1 -> mux94/2, addsub92/1
  mux57/1 -> mux59/2, addsub57/1
  mux89/1 -> mux91/2, addsub89/1
  rela89/1 -> mux89/1
  rela69/1 -> mux69/1
  rela63/1 -> mux63/1
  rela84/1 -> mux84/1
  addsub88/1 -> mux90/3
  mux83/1 -> mux85/2, addsub83/1
  rela95/1 -> mux95/1
  mux80/1 -> mux82/2, addsub80/1
  mux86/1 -> mux88/2, addsub86/1
  rela88/1 -> mux88/1
  rela62/1 -> mux62/1
  logi_b36/1 -> rela74/2, rela73/2
  mux67/1 -> mux69/2, addsub67/1
  addsub90/1 -> mux92/3
  addsub75/1 -> mux77/3
  logi_b40/1 -> rela82/2, rela81/2
  addsub87/1 -> mux89/3
  mux88/1 -> mux90/2, addsub88/1
  logi_b39/1 -> rela80/2, rela79/2
  logi_b41/1 -> rela84/2, rela83/2
  rela70/1 -> mux70/1
  addsub83/1 -> mux85/3
  rela93/1 -> mux93/1
  mux65/1 -> mux67/2, addsub65/1
  addsub58/1 -> mux60/3
  addsub84/1 -> mux86/3
  mux70/1 -> mux72/2, addsub70/1
  addsub55/1 -> mux57/3
  addsub71/1 -> mux73/3
  rela92/1 -> mux92/1
  mux68/1 -> mux70/2, addsub68/1
  mux87/1 -> mux89/2, addsub87/1
  logi_b35/1 -> rela72/2, rela71/2
  addsub56/1 -> mux58/3
  rela81/1 -> mux81/1
  addsub72/1 -> mux74/3
  mux95/1 -> mux97/2, addsub95/1
  rela71/1 -> mux71/1
  rela83/1 -> mux83/1
  rela57/1 -> mux57/1
  rela67/1 -> mux67/1
  addsub92/1 -> mux94/3
  addsub77/1 -> mux79/3
  rela78/1 -> mux78/1
  mux71/1 -> mux73/2, addsub71/1
  rela87/1 -> mux87/1
  rela80/1 -> mux80/1
  mux76/1 -> mux78/2, addsub76/1
  logi_b28/1 -> rela58/2, rela57/2
  logi_b46/1 -> rela94/2, rela93/2
  rela73/1 -> mux73/1
  logi_b42/1 -> rela86/2, rela85/2
  addsub94/1 -> mux96/3
  mux60/1 -> mux62/2, addsub60/1
  addsub67/1 -> mux69/3
  mux69/1 -> mux71/2, addsub69/1
  mux61/1 -> mux63/2, addsub61/1
  addsub61/1 -> mux63/3
  mux85/1 -> mux87/2, addsub85/1
  addsub60/1 -> mux62/3
  logi_b44/1 -> rela90/2, rela89/2
  rela65/1 -> mux65/1
  logi_b32/1 -> rela66/2, rela65/2
  mux91/1 -> mux93/2, addsub91/1
  mux59/1 -> mux61/2, addsub59/1
  logi_b43/1 -> rela88/2, rela87/2
  addsub81/1 -> mux83/3
  mux78/1 -> mux80/2, addsub78/1
  addsub86/1 -> mux88/3
  mux77/1 -> mux79/2, addsub77/1
  rela58/1 -> mux58/1
  rela66/1 -> mux66/1
  mux64/1 -> mux66/2, addsub64/1
  rela98/1 -> mux98/1
  mux79/1 -> mux81/2, addsub79/1
  mux81/1 -> mux83/2, addsub81/1
  addsub68/1 -> mux70/3
  mux66/1 -> mux68/2, addsub66/1
  mux72/1 -> mux74/2, addsub72/1
  mux75/1 -> mux77/2, addsub75/1
  mux73/1 -> mux75/2, addsub73/1
  addsub82/1 -> mux84/3
  addsub73/1 -> mux75/3
  rela77/1 -> mux77/1
  rela76/1 -> mux76/1
  addsub79/1 -> mux81/3
  rela82/1 -> mux82/1
  addsub76/1 -> mux78/3
  mux82/1 -> mux84/2, addsub82/1
  logi_b38/1 -> rela78/2, rela77/2
  rela74/1 -> mux74/1
  logi_b37/1 -> rela76/2, rela75/2
  addsub78/1 -> mux80/3
  rela75/1 -> mux75/1
  rela85/1 -> mux85/1
  mux84/1 -> mux86/2, addsub84/1
  addsub85/1 -> mux87/3
  rela61/1 -> mux61/1
  logi_b34/1 -> rela70/2, rela69/2
  mux62/1 -> mux64/2, addsub62/1
  mux58/1 -> mux60/2, addsub58/1
  logi_b29/1 -> rela60/2, rela59/2
  mux63/1 -> mux65/2, addsub63/1
  mux74/1 -> mux76/2, addsub74/1
  logi_b33/1 -> rela68/2, rela67/2
  rela90/1 -> mux90/1
  mux55/1 -> mux57/2, addsub55/1
  addsub64/1 -> mux66/3
  logi_b31/1 -> rela64/2, rela63/2
  mux56/1 -> mux58/2, addsub56/1
  addsub65/1 -> mux67/3
  rela72/1 -> mux72/1
  rela64/1 -> mux64/1
  Scaling/1 -> Gate_out1/1
  Slice2/1 -> AddSub20/2
  AddSub201/1 -> Mux100/3
  Mux114/1 -> AddSub118/1, Delay591/1
  logi_b56/1 -> Relational129/2, Relational185/2
  logi_b84/1 -> Relational162/2, Relational175/2
  AddSub161/1 -> Mux172/3
  Delay335/1 -> Mux143/1
  logi_b83/1 -> Relational183/2, Relational106/2
  addsub101/1 -> mux103/3
  Relational159/1 -> Delay367/1
  Delay453/1 -> Mux100/2
  addsub102/1 -> mux104/3
  Relational164/1 -> Delay397/1
  AddSub193/1 -> Mux192/3
  Delay563/1 -> Mux132/1
  Delay224/1 -> Mux112/1
  Relational118/1 -> Delay229/1
  Delay440/1 -> Mux196/2
  AddSub101/1 -> Mux105/3
  Delay466/1 -> Mux173/2
  Delay376/1 -> Mux145/2
  Relational131/1 -> Delay548/1
  Delay235/1 -> Mux194/1
  Relational117/1 -> Delay596/1
  logi_b66/1 -> Relational120/2, Relational137/2
  mux111/1 -> AddSub161/1, Delay451/1
  AddSub119/1 -> Mux116/3
  AddSub102/1 -> Mux200/3
  Delay347/1 -> Mux110/2
  Delay254/1 -> Mux149/1
  logi_b60/1 -> Relational112/2, Relational118/2
  Delay464/1 -> Relational177/1, Delay467/1
  AddSub152/1 -> Mux148/3
  Relational102/1 -> Delay448/1
  Delay226/1 -> Mux104/2
  Delay233/1 -> Mux137/1
  Delay424/1 -> Relational202/1, Delay428/1
  Delay351/1 -> Mux151/2
  Delay549/1 -> Mux126/2
  adsbu105/1 -> mux107/3
  Mux181/1 -> AddSub186/1, Delay391/1
  AddSub190/1 -> Mux189/3
  Relational183/1 -> Delay482/1
  logi_b94/1 -> Relational195/2, Relational194/2
  logi_b95/1 -> Relational197/2, Relational200/2
  Delay368/1 -> Mux156/2
  Relational192/1 -> Delay409/1
  Delay469/1 -> Mux174/2
  Mux136/1 -> AddSub142/1, Delay248/1
  Delay373/1 -> Mux144/2
  AddSub169/1 -> Mux167/3
  Delay364/1 -> Mux155/1
  Delay359/1 -> Delay363/1, Relational158/1
  mux112/1 -> AddSub127/1, Delay545/1
  Delay421/1 -> Mux163/1
  Delay411/1 -> Mux191/2
  AddSub137/1 -> Mux136/3
  Relational190/1 -> Delay508/1
  Delay491/1 -> Mux184/2
  logi_b89/1 -> Relational169/2, Relational187/2
  Mux186/1 -> AddSub188/1, Delay502/1
  logi_b62/1 -> Relational114/2, Relational133/2
  Delay493/1 -> Mux185/1
  Delay520/1 -> Delay523/1, Relational170/1
  AddSub151/1 -> Mux147/3
  Delay443/1 -> Mux197/2
  AddSub184/1 -> Mux181/3
  Delay427/1 -> Mux199/2
  Delay255/1 -> Mux149/2
  Relational114/1 -> Delay585/1
  logi_b79/1 -> Relational178/2, Relational201/2
  logi_b64/1 -> Relational116/2, Relational135/2
  AddSub155/1 -> Mux153/3
  Delay494/1 -> Mux185/2
  Delay379/1 -> Mux146/1
  AddSub164/1 -> Mux162/3
  AddSub171/1 -> Mux169/3
  AddSub166/1 -> Mux164/3
  Mux163/1 -> AddSub196/1, Delay427/1
  Relational157/1 -> Delay361/1
  Mux125/1 -> AddSub129/1, Delay549/1
  Delay213/1 -> Mux111/2
  Constant7/1 -> addsub20/2, addsub38/2, addsub72/2, addsub90/2, addsub100/2, AddSub114/2, AddSub145/2, AddSub166/2, AddSub197/2, AddSub236/2, AddSub298/2, AddSub297/2, AddSub296/2, AddSub295/2, AddSub290/2, AddSub284/2, AddSub282/2, AddSub269/2, AddSub268/2, AddSub267/2, AddSub266/2, AddSub265/2, AddSub264/2, AddSub210/2, AddSub279/2, AddSub277/2, AddSub276/2, AddSub275/2, AddSub274/2, AddSub273/2, AddSub272/2, AddSub257/2, AddSub252/2, AddSub250/2, AddSub249/2, AddSub138/2, AddSub200/2, AddSub199/2, AddSub198/2, AddSub192/2, AddSub186/2, AddSub184/2, AddSub171/2, AddSub170/2, AddSub169/2, AddSub168/2, AddSub167/2, AddSub107/2, AddSub181/2, AddSub179/2, AddSub178/2, AddSub177/2, AddSub176/2, AddSub175/2, AddSub174/2, AddSub159/2, AddSub154/2, AddSub152/2, AddSub151/2, AddSub149/2, AddSub148/2, AddSub147/2, AddSub146/2, AddSub141/2, AddSub133/2, AddSub131/2, AddSub119/2, AddSub118/2, AddSub117/2, AddSub116/2, AddSub115/2, AddSub183/2, AddSub129/2, AddSub127/2, addsub110/2, addsub108/2, addsub106/2, addsub104/2, addsub102/2, addsub98/2, addsub96/2, addsub94/2, addsub92/2, addsub88/2, addsub86/2, addsub84/2, addsub82/2, addsub80/2, addsub78/2, addsub76/2, addsub74/2, addsub70/2, addsub68/2, addsub66/2, addsub64/2, addsub62/2, addsub60/2, addsub58/2, addsub56/2, addsub54/2, addsub52/2, addsub50/2, addsub48/2, addsub46/2, addsub44/2, addsub42/2, addsub40/2, addsub36/2, addsub34/2, addsub32/2, addsub30/2, addsub28/2, addsub26/2, addsub24/2, addsub22/2, addsub18/2, addsub16/2, addsub14/2, addsub12/2, addsub10/2, addsub8/2, addsub6/2, addsub4/2, addsub2/2, mux2/3
  Delay406/1 -> Mux192/1
  mux109/1 -> mux111/2, addsub109/1
  Delay558/1 -> Mux105/2
  Delay253/1 -> Mux140/2
  Mux158/1 -> Delay389/1, AddSub163/1
  Delay410/1 -> Mux191/1
  Mux100/1 -> AddSub103/1, Delay456/1
  Delay471/1 -> Delay475/1, Relational180/1
  Delay576/1 -> Relational142/1, Delay246/1
  mux100/1 -> mux102/2, addsub100/1
  Relational187/1 -> Delay498/1
  Delay407/1 -> Mux192/2
  Delay225/1 -> Mux104/1
  Mux171/1 -> AddSub175/1, Delay466/1
  rela103/1 -> mux103/1
  Mux177/1 -> AddSub181/1, Delay483/1
  Relational201/1 -> Delay433/1
  logi_b85/1 -> Relational165/2, Relational164/2
  Delay403/1 -> Mux103/2
  Delay417/1 -> Mux159/1
  Delay229/1 -> Mux105/1
  AddSub162/1 -> Mux96/3
  logi_b59/1 -> Relational111/2, Relational105/2
  Relational188/1 -> Delay501/1
  AddSub114/1 -> Mux111/3
  Delay523/1 -> Delay526/1, Relational171/1
  addsub103/1 -> mux105/3
  AddSub117/1 -> Mux114/3
  Delay365/1 -> Mux155/2
  Mux105/1 -> AddSub105/1, Delay561/1
  Delay445/1 -> Delay447/1, Relational102/1
  Mux115/1 -> AddSub119/1, Delay594/1
  Relational148/1 -> Delay379/1
  Delay348/1 -> Relational154/1, Delay352/1
  Delay509/1 -> Mux189/2
  Relational195/1 -> Delay412/1
  Delay418/1 -> Mux159/2
  AddSub199/1 -> Mux196/3
  Mux154/1 -> AddSub157/1, Delay365/1
  Delay234/1 -> Mux137/2
  Relational153/1 -> Delay254/1
  rela111/1 -> mux111/1
  AddSub158/1 -> Mux156/3
  Delay370/1 -> Relational146/1, Delay374/1
  mux106/1 -> mux108/2, addsub106/1
  mux101/1 -> mux103/2, addsub101/1
  Relational143/1 -> Delay336/1
  Delay470/1 -> Delay471/1, Relational179/1
  Delay580/1 -> Mux112/2
  Delay419/1 -> Mux180/2
  Delay486/1 -> Relational165/1, Delay395/1
  Delay366/1 -> Relational161/1, Delay341/1
  Mux160/1 -> AddSub164/1, Delay488/1
  Mux190/1 -> AddSub191/1, Delay449/1
  Relational186/1 -> Delay493/1
  AddSub185/1 -> Mux185/3
  Mux200/1 -> AddSub140/1, Delay232/1
  Delay385/1 -> Relational153/1, Delay388/1
  AddSub187/1 -> Mux186/3
  Delay513/1 -> Mux166/2
  Delay504/1 -> Mux188/1
  Delay390/1 -> Mux182/1
  logi_b65/1 -> Relational117/2, Relational136/2
  Relational202/1 -> Delay426/1
  Delay468/1 -> Mux174/1
  Relational168/1 -> Delay515/1
  Delay409/1 -> Mux180/1
  AddSub174/1 -> Mux171/3
  addsub108/1 -> mux110/3
  Mux129/1 -> AddSub133/1, Delay211/1
  Delay518/1 -> Delay520/1, Relational169/1
  Mux194/1 -> Delay213/1, AddSub114/1
  Mux101/1 -> AddSub106/1, Delay459/1
  Relational140/1 -> Delay252/1
  Delay527/1 -> Mux181/1
  Delay598/1 -> Relational140/1, Delay250/1
  AddSub156/1 -> Mux154/3
  Mux102/1 -> AddSub182/1, Delay485/1
  Relational177/1 -> Delay465/1
  Relational184/1 -> Delay490/1
  AddSub179/1 -> Mux177/3
  Delay481/1 -> Relational162/1, Delay486/1
  Delay381/1 -> Delay385/1, Relational150/1
  Mux172/1 -> AddSub172/1, Delay484/1
  Relational120/1 -> Delay210/1
  Mux183/1 -> AddSub130/1, Delay550/1
  AddSub191/1 -> Mux198/3
  Mux159/1 -> AddSub195/1, Delay423/1
  Mux149/1 -> AddSub159/1, Delay346/1
  Delay568/1 -> Mux133/1
  mux99/1 -> mux101/2, addsub99/1
  Delay246/1 -> Relational143/1, Delay339/1
  Delay505/1 -> Mux188/2
  logi_b93/1 -> Relational191/2, Relational193/2
  Delay228/1 -> Delay559/1, Relational118/1
  Relational178/1 -> Delay468/1
  Delay562/1 -> Relational133/1, Delay565/1
  Delay448/1 -> Mux198/1
  Delay355/1 -> Delay356/1, Relational156/1
  mux105/1 -> mux107/2, adsbu105/1
  AddSub196/1 -> Mux199/3
  Mux116/1 -> AddSub131/1, Delay597/1
  Delay451/1 -> Mux172/2
  Relational104/1 -> Delay455/1
  Delay567/1 -> Delay570/1, Relational135/1
  Relational191/1 -> Delay410/1
  Delay346/1 -> Mux157/2
  Delay245/1 -> Mux194/2
  Delay575/1 -> Mux135/2
  Relational175/1 -> Delay461/1
  Delay551/1 -> Relational111/1, Delay223/1
  Delay425/1 -> Relational201/1, Delay445/1
  Mux157/1 -> Delay463/1, AddSub174/1
  Delay455/1 -> Mux101/1
  AddSub175/1 -> Mux173/3
  Delay447/1 -> Delay450/1, Relational103/1
  Delay353/1 -> Mux152/1
  Delay502/1 -> Mux187/2
  logi_b77/1 -> Relational176/2, Relational182/2
  AddSub113/1 -> Mux160/3
  logi_b87/1 -> Relational167/2, Relational184/2
  Delay510/1 -> Mux165/2
  AddSub186/1 -> Mux182/3
  rela109/1 -> mux109/1
  Delay482/1 -> Mux178/1
  Delay503/1 -> Relational190/1, Delay507/1
  AddSub132/1 -> Mux132/3
  Relational149/1 -> Delay383/1
  logi_b63/1 -> Relational115/2, Relational134/2
  logi_b52/1 -> rela106/2, rela105/2
  Delay387/1 -> Mux148/2
  AddSub176/1 -> Mux174/3
  AddSub146/1 -> Mux143/3
  AddSub170/1 -> Mux168/3
  Delay472/1 -> Mux175/1
  Delay352/1 -> Relational155/1, Delay355/1
  rela110/1 -> mux110/1
  Relational160/1 -> Delay345/1
  Delay250/1 -> Relational144/1, Delay334/1
  AddSub159/1 -> Mux157/3
  AddSub177/1 -> Mux175/3
  Relational198/1 -> Delay438/1
  Delay487/1 -> Mux171/1
  Delay476/1 -> Mux176/1
  Delay211/1 -> Mux130/2
  AddSub153/1 -> Mux152/3
  Delay595/1 -> Relational120/1, Delay598/1
  Delay452/1 -> Mux100/1
  Delay446/1 -> Mux172/1
  Relational200/1 -> Delay421/1
  Delay449/1 -> Mux198/2
  Relational166/1 -> Delay396/1
  Delay572/1 -> Mux134/2
  Delay454/1 -> Relational106/1, Delay457/1
  Delay383/1 -> Mux147/1
  Mux176/1 -> AddSub179/1, Delay480/1
  logi_b55/1 -> rela112/2, rela111/2
  Mux143/1 -> AddSub147/1, Delay373/1
  Mux169/1 -> AddSub184/1, Delay529/1
  Delay336/1 -> Mux96/1
  Delay507/1 -> Relational193/1, Delay405/1
  Relational197/1 -> Delay416/1
  Mux148/1 -> AddSub154/1, Delay255/1
  AddSub194/1 -> Mux104/3
  Mux142/1 -> AddSub146/1, Delay369/1
  logi_b61/1 -> Relational113/2, Relational132/2
  Delay460/1 -> Relational164/1, Delay399/1
  Relational165/1 -> Delay392/1
  Delay475/1 -> Delay478/1, Relational181/1
  Delay483/1 -> Mux178/2
  Relational105/1 -> Delay225/1
  Delay232/1 -> Mux138/2
  Relational122/1 -> Delay506/1
  mux108/1 -> mux110/2, addsub108/1
  AddSub148/1 -> Mux145/3
  Mux141/1 -> Delay337/1, AddSub162/1
  AddSub141/1 -> Mux140/3
  Delay584/1 -> Relational114/1, Delay587/1
  Mux103/1 -> Delay394/1, AddSub166/1
  addsub109/1 -> mux111/3
  Mux189/1 -> AddSub193/1, Delay407/1
  logi_b73/1 -> Relational149/2, Relational157/2
  mux107/1 -> mux109/2, addsub107/1
  Delay530/1 -> Relational191/1, Delay408/1
  rela107/1 -> mux107/1
  logi_b91/1 -> Relational171/2, Relational189/2
  Mux193/1 -> AddSub198/1, Delay435/1
  logi_b82/1 -> Relational181/2, Relational104/2
  Mux180/1 -> AddSub180/1, Delay437/1
  Delay574/1 -> Mux135/1
  Mux185/1 -> AddSub187/1, Delay499/1
  Delay345/1 -> Mux157/1
  AddSub167/1 -> Mux165/3
  rela106/1 -> mux106/1
  logi_b90/1 -> Relational170/2, Relational188/2
  Mux188/1 -> AddSub190/1, Delay509/1
  AddSub178/1 -> Mux176/3
  Delay508/1 -> Mux189/1
  Delay212/1 -> Mux111/1
  Delay426/1 -> Mux199/1
  Delay581/1 -> Relational113/1, Delay584/1
  Relational142/1 -> Delay247/1
  Delay412/1 -> Mux193/1
  logi_b54/1 -> rela110/2, rela109/2
  Mux111/1 -> AddSub115/1, Delay580/1
  Mux96/1 -> AddSub143/1, Delay347/1
  logi_b50/1 -> rela102/2, rela101/2
  rela105/1 -> mux105/1
  Relational103/1 -> Delay452/1
  Delay431/1 -> Mux200/2
  AddSub145/1 -> Mux142/3
  Delay392/1 -> Mux164/1
  logi_b58/1 -> Relational98/2, Relational122/2
  Relational111/1 -> Delay212/1
  Mux195/1 -> AddSub199/1, Delay440/1
  Delay405/1 -> Relational194/1, Delay420/1
  AddSub142/1 -> Mux141/3
  Delay565/1 -> Delay567/1, Relational134/1
  Delay369/1 -> Mux143/2
  Delay433/1 -> Mux190/1
  Delay501/1 -> Mux187/1
  Relational139/1 -> Delay233/1
  Mux167/1 -> AddSub170/1, Delay522/1
  Delay465/1 -> Mux173/1
  Delay231/1 -> Mux138/1
  Delay479/1 -> Mux177/1
  AddSub138/1 -> Mux137/3
  Relational156/1 -> Delay357/1
  AddSub157/1 -> Mux155/3
  logical_x0/1 -> Delay543/1, Relational129/1, rela112/1, rela110/1, rela108/1, rela106/1, rela104/1, rela102/1, rela100/1, rela98/1, rela96/1, rela94/1, rela92/1, rela90/1, rela88/1, rela86/1, rela84/1, rela82/1, rela80/1, rela78/1, rela76/1, rela74/1, rela72/1, rela70/1, rela68/1, rela66/1, rela64/1, rela62/1, rela60/1, rela58/1, rela56/1, rela54/1, rela52/1, rela50/1, rela48/1, rela46/1, rela44/1, rela42/1, rela40/1, rela38/1, rela36/1, rela34/1, rela32/1, rela30/1, rela28/1, rela26/1, rela24/1, rela22/1, rela20/1, rela18/1, rela16/1, rela14/1, rela12/1, rela10/1, rela8/1, rela6/1, rela4/1, rela2/1
  AddSub143/1 -> Mux110/3
  Delay372/1 -> Mux144/1
  Delay450/1 -> Delay454/1, Relational104/1
  Delay252/1 -> Mux140/1
  rela104/1 -> mux104/1
  Delay357/1 -> Mux153/1
  Delay485/1 -> Mux179/2
  Mux198/1 -> AddSub201/1, Delay453/1
  Delay546/1 -> Relational98/1, Delay551/1
  mux103/1 -> mux105/2, addsub103/1
  logi_b98/1 -> Relational139/2, Relational138/2
  Relational180/1 -> Delay476/1
  Delay344/1 -> Delay464/1, Relational176/1
  Delay400/1 -> Mux162/1
  Delay395/1 -> Delay511/1, Relational166/1
  Delay514/1 -> Relational168/1, Delay518/1
  Mux145/1 -> AddSub149/1, Delay380/1
  Mux196/1 -> AddSub200/1, Delay443/1
  Mux155/1 -> AddSub158/1, Delay368/1
  AddSub103/1 -> Mux101/3
  Delay399/1 -> Delay489/1, Relational172/1
  Mux152/1 -> AddSub155/1, Delay358/1
  Delay561/1 -> Mux131/2
  Delay548/1 -> Mux126/1
  AddSub183/1 -> Mux194/3
  Delay401/1 -> Relational192/1, Delay425/1
  Delay499/1 -> Mux186/2
  Delay545/1 -> Mux125/2
  Delay474/1 -> Mux175/2
  Delay332/1 -> Mux142/1
  Relational182/1 -> Delay519/1
  Delay461/1 -> Mux179/1
  AddSub129/1 -> Mux126/3
  Delay495/1 -> Relational105/1, Delay228/1
  mux104/1 -> mux106/2, addsub104/1
  AddSub115/1 -> Mux112/3
  Delay543/1 -> Relational131/1, Delay546/1
  Delay498/1 -> Mux186/1
  Delay389/1 -> Mux170/2
  Mux110/1 -> AddSub144/1, Delay351/1
  Delay361/1 -> Mux154/1
  addsub110/1 -> mux112/3
  Mux179/1 -> Delay398/1, AddSub113/1
  Delay416/1 -> Mux195/1
  Delay463/1 -> Mux171/2
  Delay343/1 -> Mux158/2
  Delay596/1 -> Mux129/1
  Mux147/1 -> AddSub152/1, Delay387/1
  Delay490/1 -> Mux184/1
  Delay396/1 -> Mux165/1
  Mux165/1 -> AddSub168/1, Delay513/1
  AddSub168/1 -> Mux166/3
  Mux199/1 -> AddSub102/1, Delay431/1
  AddSub198/1 -> Mux195/3
  Delay521/1 -> Mux168/1
  AddSub135/1 -> Mux134/3
  Delay560/1 -> Mux131/1
  logi_b72/1 -> Relational148/2, Relational156/2
  logi_b97/1 -> Relational199/2, Relational101/2
  Relational158/1 -> Delay364/1
  Relational167/1 -> Delay512/1
  Delay597/1 -> Mux129/2
  Delay582/1 -> Mux113/1
  Relational179/1 -> Delay472/1
  AddSub192/1 -> Mux191/3
  rela112/1 -> mux112/1
  Delay435/1 -> Mux195/2
  Delay437/1 -> Mux190/2
  AddSub130/1 -> Mux127/3
  Delay374/1 -> Relational147/1, Delay377/1
  Delay512/1 -> Mux166/1
  AddSub105/1 -> Mux131/3
  Delay398/1 -> Mux160/2
  Relational196/1 -> Delay473/1
  Relational155/1 -> Delay353/1
  logi_b96/1 -> Relational198/2, Relational202/2
  Mux178/1 -> AddSub107/1, Delay403/1
  AddSub182/1 -> Mux179/3
  Delay342/1 -> Mux158/1
  Relational170/1 -> Delay524/1
  Delay578/1 -> Mux136/1
  rela108/1 -> mux108/1
  Delay571/1 -> Mux134/1
  Relational132/1 -> Delay560/1
  Relational181/1 -> Delay479/1
  Relational169/1 -> Delay521/1
  Delay339/1 -> Delay348/1, Relational151/1
  AddSub173/1 -> Mux180/3
  Relational135/1 -> Delay571/1
  Relational134/1 -> Delay568/1
  AddSub160/1 -> Mux158/3
  Mux164/1 -> AddSub167/1, Delay510/1
  AddSub197/1 -> Mux193/3
  Relational98/1 -> Delay235/1
  Delay579/1 -> Mux136/2
  Relational194/1 -> Delay417/1
  Delay524/1 -> Mux169/1
  Delay408/1 -> Relational195/1, Delay415/1
  logi_b53/1 -> rela108/2, rela107/2
  Delay516/1 -> Mux167/2
  logi_b81/1 -> Relational180/2, Relational103/2
  AddSub104/1 -> Mux159/3
  Delay391/1 -> Mux182/2
  Delay356/1 -> Delay359/1, Relational157/1
  Delay593/1 -> Mux116/1
  Delay564/1 -> Mux132/2
  Relational101/1 -> Delay430/1
  Delay506/1 -> Mux127/1
  Delay456/1 -> Mux101/2
  logi_b57/1 -> Relational131/2, Relational196/2
  logi_b88/1 -> Relational168/2, Relational186/2
  Delay438/1 -> Mux196/1
  Delay384/1 -> Mux147/2
  Delay340/1 -> Mux110/1
  Relational161/1 -> Delay342/1
  Mux134/1 -> AddSub136/1, Delay575/1
  Mux175/1 -> AddSub178/1, Delay477/1
  Relational173/1 -> Delay390/1
  AddSub131/1 -> Mux129/3
  Delay526/1 -> Relational173/1, Delay530/1
  Delay247/1 -> Mux141/1
  Delay341/1 -> Delay401/1, Relational182/1
  Mux166/1 -> AddSub169/1, Delay516/1
  Relational116/1 -> Delay593/1
  logi_b68/1 -> Relational144/2, Relational143/2
  Mux140/1 -> Delay333/1, AddSub145/1
  Delay380/1 -> Mux146/2
  logi_b74/1 -> Relational150/2, Relational158/2
  Delay375/1 -> Mux145/1
  AddSub189/1 -> Mux188/3
  Mux174/1 -> AddSub177/1, Delay474/1
  Delay337/1 -> Mux96/2
  addsub100/1 -> mux102/3
  Delay489/1 -> Relational184/1, Delay492/1
  AddSub163/1 -> Mux170/3
  Mux144/1 -> AddSub148/1, Delay376/1
  Delay586/1 -> Mux114/2
  Delay397/1 -> Mux160/1
  mux110/1 -> mux112/2, addsub110/1
  Mux126/1 -> AddSub183/1, Delay245/1
  Delay529/1 -> Mux181/2
  Delay525/1 -> Mux169/2
  Delay550/1 -> Mux127/2
  Delay354/1 -> Mux152/2
  Delay248/1 -> Mux141/2
  Relational154/1 -> Delay350/1
  Relational199/1 -> Delay442/1
  AddSub181/1 -> Mux178/3
  Delay458/1 -> Mux102/1
  Delay377/1 -> Delay378/1, Relational148/1
  Delay388/1 -> Relational160/1, Delay344/1
  addsub106/1 -> mux108/3
  Relational189/1 -> Delay504/1
  logi_b69/1 -> Relational145/2, Relational151/2
  Delay362/1 -> Mux154/2
  Delay378/1 -> Delay381/1, Relational149/1
  Delay473/1 -> Mux183/1
  AddSub188/1 -> Mux187/3
  Delay423/1 -> Mux163/2
  addsub99/1 -> mux101/3
  Mux162/1 -> AddSub165/1, Delay491/1
  Mux173/1 -> AddSub176/1, Delay469/1
  logi_b75/1 -> Relational153/2, Relational159/2
  Delay428/1 -> Relational101/1, Delay432/1
  Relational150/1 -> Delay386/1
  Delay480/1 -> Mux177/2
  Delay585/1 -> Mux114/1
  logi_b78/1 -> Relational177/2, Relational192/2
  Delay570/1 -> Delay573/1, Relational136/1
  Mux182/1 -> AddSub192/1, Delay411/1
  AddSub195/1 -> Mux163/3
  Relational115/1 -> Delay590/1
  Relational137/1 -> Delay578/1
  Relational185/1 -> Delay446/1
  mux102/1 -> mux104/2, addsub102/1
  logi_b71/1 -> Relational147/2, Relational155/2
  Delay590/1 -> Mux115/1
  Delay210/1 -> Mux130/1
  Mux153/1 -> AddSub156/1, Delay362/1
  Delay415/1 -> Delay436/1, Relational197/1
  Delay511/1 -> Relational167/1, Delay514/1
  Delay484/1 -> Mux183/2
  Delay492/1 -> Relational186/1, Delay496/1
  Relational171/1 -> Delay527/1
  rela101/1 -> mux101/1
  AddSub106/1 -> Mux102/3
  Delay358/1 -> Mux153/2
  Delay589/1 -> Delay592/1, Relational116/1
  Delay350/1 -> Mux151/1
  AddSub200/1 -> Mux197/3
  Delay420/1 -> Delay424/1, Relational200/1
  logi_b76/1 -> Relational160/2, Relational161/2
  Relational151/1 -> Delay340/1
  logi_b70/1 -> Relational146/2, Relational154/2
  AddSub107/1 -> Mux103/3
  logi_b67/1 -> Relational140/2, Relational142/2
  Delay367/1 -> Mux156/1
  Mux168/1 -> AddSub171/1, Delay525/1
  AddSub154/1 -> Mux149/3
  Relational146/1 -> Delay372/1
  Delay442/1 -> Mux197/1
  Mux133/1 -> AddSub135/1, Delay572/1
  Delay414/1 -> Mux193/2
  Mux170/1 -> AddSub173/1, Delay419/1
  Relational147/1 -> Delay375/1
  Mux104/1 -> AddSub101/1, Delay558/1
  AddSub180/1 -> Mux190/3
  Mux192/1 -> Delay418/1, AddSub104/1
  Mux113/1 -> AddSub117/1, Delay586/1
  AddSub134/1 -> Mux133/3
  Delay583/1 -> Mux113/2
  Delay569/1 -> Mux133/2
  AddSub118/1 -> Mux115/3
  Relational176/1 -> Delay487/1
  Delay559/1 -> Relational132/1, Delay562/1
  Mux131/1 -> AddSub132/1, Delay564/1
  Delay457/1 -> Relational175/1, Delay460/1
  Relational112/1 -> Delay224/1
  Delay436/1 -> Relational198/1, Delay441/1
  Delay394/1 -> Mux164/2
  Relational133/1 -> Delay563/1
  Delay591/1 -> Mux115/2
  Delay500/1 -> Delay503/1, Relational189/1
  Delay496/1 -> Delay497/1, Relational187/1
  Delay587/1 -> Delay589/1, Relational115/1
  AddSub136/1 -> Mux135/3
  logi_b92/1 -> Relational173/2, Relational190/2
  Delay515/1 -> Mux167/1
  Delay459/1 -> Mux102/2
  Relational162/1 -> Delay402/1
  Relational144/1 -> Delay332/1
  Mux187/1 -> AddSub189/1, Delay505/1
  Delay488/1 -> Mux162/2
  Delay223/1 -> Delay581/1, Relational112/1
  Relational113/1 -> Delay582/1
  addsub104/1 -> mux106/3
  Delay467/1 -> Relational178/1, Delay470/1
  Mux156/1 -> AddSub160/1, Delay343/1
  rela102/1 -> mux102/1
  Delay594/1 -> Mux116/2
  Delay439/1 -> Relational196/1, Delay462/1
  Relational193/1 -> Delay406/1
  AddSub116/1 -> Mux113/3
  Delay592/1 -> Delay595/1, Relational117/1
  Relational136/1 -> Delay574/1
  Delay462/1 -> Relational122/1, Delay495/1
  Mux197/1 -> AddSub138/1, Delay234/1
  Mux184/1 -> AddSub185/1, Delay494/1
  Mux130/1 -> AddSub141/1, Delay253/1
  Mux146/1 -> AddSub151/1, Delay384/1
  Mux191/1 -> Delay414/1, AddSub197/1
  Delay573/1 -> Relational137/1, Delay576/1
  Delay519/1 -> Mux170/1
  Delay334/1 -> Delay370/1, Relational145/1
  Relational145/1 -> Delay335/1
  AddSub133/1 -> Mux130/3
  Delay544/1 -> Mux125/1
  AddSub127/1 -> Mux125/3
  logi_b80/1 -> Relational179/2, Relational102/2
  Delay478/1 -> Relational183/1, Delay481/1
  logi_b51/1 -> rela103/2, rela104/2
  Delay497/1 -> Delay500/1, Relational188/1
  addsub107/1 -> mux109/3
  Relational129/1 -> Delay544/1
  AddSub140/1 -> Mux138/3
  Mux132/1 -> AddSub134/1, Delay569/1
  Mux135/1 -> AddSub137/1, Delay579/1
  AddSub165/1 -> Mux184/3
  Mux112/1 -> AddSub116/1, Delay583/1
  Mux127/1 -> Delay226/1, AddSub194/1
  logi_b86/1 -> Relational166/2, Relational172/2
  Delay402/1 -> Mux103/1
  Relational172/1 -> Delay400/1
  Delay386/1 -> Mux148/1
  Relational106/1 -> Delay458/1
  Delay363/1 -> Relational159/1, Delay366/1
  Mux151/1 -> AddSub153/1, Delay354/1
  AddSub147/1 -> Mux144/3
  Delay477/1 -> Mux176/2
  AddSub144/1 -> Mux151/3
  Relational138/1 -> Delay231/1
  AddSub172/1 -> Mux183/3
  Delay430/1 -> Mux200/1
  logical_y0/1 -> Delay439/1, Relational185/1, rela111/1, rela109/1, rela107/1, rela105/1, rela103/1, rela101/1, rela99/1, rela97/1, rela95/1, rela93/1, rela91/1, rela89/1, rela87/1, rela85/1, rela83/1, rela81/1, rela79/1, rela77/1, rela75/1, rela73/1, rela71/1, rela69/1, rela67/1, rela65/1, rela63/1, rela61/1, rela59/1, rela57/1, rela55/1, rela53/1, rela51/1, rela49/1, rela47/1, rela45/1, rela43/1, rela41/1, rela39/1, rela37/1, rela35/1, rela33/1, rela31/1, rela29/1, rela27/1, rela25/1, rela23/1, rela21/1, rela19/1, rela17/1, rela15/1, rela13/1, rela11/1, rela9/1, rela7/1, rela5/1, rela3/1, rela1/1
  AddSub149/1 -> Mux146/3
  Constant2/1 -> addsub17/2, addsub19/2, addsub23/2, addsub25/2, addsub27/2, addsub29/2, addsub31/2, addsub37/2, addsub41/2, addsub43/2, addsub45/2, addsub47/2, addsub49/2, addsub53/2, addsub69/2, addsub71/2, addsub75/2, addsub77/2, addsub79/2, addsub81/2, addsub83/2, addsub89/2, AddSub130/2, AddSub194/2, AddSub105/2, AddSub132/2, AddSub134/2, AddSub135/2, AddSub136/2, AddSub162/2, AddSub144/2, AddSub153/2, AddSub155/2, AddSub156/2, AddSub157/2, AddSub160/2, AddSub182/2, AddSub113/2, AddSub165/2, AddSub185/2, AddSub187/2, AddSub188/2, AddSub189/2, AddSub104/2, AddSub196/2, AddSub238/2, AddSub205/2, AddSub294/2, AddSub293/2, AddSub207/2, AddSub291/2, AddSub288/2, AddSub287/2, AddSub286/2, AddSub285/2, AddSub283/2, AddSub263/2, AddSub262/2, AddSub211/2, AddSub280/2, AddSub209/2, AddSub206/2, AddSub299/2, AddSub289/2, AddSub278/2, AddSub271/2, AddSub261/2, AddSub258/2, AddSub256/2, AddSub255/2, AddSub254/2, AddSub140/2, AddSub102/2, AddSub195/2, AddSub193/2, AddSub190/2, AddSub164/2, AddSub106/2, AddSub103/2, AddSub201/2, AddSub191/2, AddSub180/2, AddSub173/2, AddSub163/2, AddSub158/2, AddSub143/2, AddSub142/2, AddSub137/2, AddSub101/2, AddSub172/2, AddSub161/2, addsub109/2, addsub107/2, adsbu105/2, addsub103/2, addsub101/2, addsub99/2, addsub97/2, addsub95/2, addsub93/2, addsub91/2, addsub87/2, addsub85/2, addsub73/2, addsub67/2, addsub65/2, addsub63/2, addsub61/2, addsub59/2, addsub57/2, addsub55/2, addsub51/2, addsub39/2, addsub35/2, addsub33/2, addsub21/2, addsub15/2, addsub13/2, addsub11/2, addsub9/2, addsub7/2, addsub5/2, addsub3/2, addsub1/2, mux1/3
  Delay522/1 -> Mux168/2
  Delay441/1 -> Relational199/1, Delay444/1
  Delay333/1 -> Mux142/2
  AddSub299/1 -> Mux204/3
  logi_b110/1 -> Relational262/2, Relational275/2
  logi_b109/1 -> Relational283/2, Relational210/2
  Delay726/1 -> Relational238/1
  Relational259/1 -> Delay661/1
  Delay747/1 -> Mux204/2
  Relational264/1 -> Delay691/1
  AddSub291/1 -> Mux292/3
  Delay734/1 -> Mux296/2
  Delay760/1 -> Mux273/2
  AddSub205/1 -> Mux300/3
  Delay624/1 -> Mux249/1
  Delay758/1 -> Relational277/1, Delay761/1
  AddSub250/1 -> Mux248/3
  Relational206/1 -> Delay742/1
  Delay613/1 -> Mux237/1
  Delay718/1 -> Relational302/1, Delay722/1
  Mux281/1 -> AddSub284/1, Delay685/1
  AddSub288/1 -> Mux289/3
  Relational283/1 -> Delay776/1
  logi_b120/1 -> Relational295/2, Relational294/2
  logi_b121/1 -> Relational297/2, Relational300/2
  Delay662/1 -> Mux256/2
  Relational292/1 -> Delay703/1
  Delay763/1 -> Mux274/2
  AddSub267/1 -> Mux267/3
  Delay658/1 -> Mux255/1
  Delay432/1 -> Relational138/1, Delay610/1
  Delay715/1 -> Mux263/1
  Delay705/1 -> Mux291/2
  Relational290/1 -> Delay802/1
  Delay785/1 -> Mux284/2
  logi_b115/1 -> Relational269/2, Relational287/2
  Mux286/1 -> AddSub286/1, Delay796/1
  Delay787/1 -> Mux285/1
  Delay814/1 -> Delay817/1, Relational270/1
  AddSub249/1 -> Mux247/3
  Delay737/1 -> Mux297/2
  AddSub282/1 -> Mux281/3
  Delay721/1 -> Mux299/2
  Delay625/1 -> Mux249/2
  logi_b105/1 -> Relational278/2, Relational301/2
  Delay788/1 -> Mux285/2
  AddSub262/1 -> Mux262/3
  AddSub269/1 -> Mux269/3
  AddSub264/1 -> Mux264/3
  Mux263/1 -> AddSub294/1, Delay721/1
  Relational203/1 -> Delay655/1
  Delay700/1 -> Mux292/1
  Mux258/1 -> Delay683/1, AddSub261/1
  Delay704/1 -> Mux291/1
  Mux204/1 -> AddSub206/1, Delay750/1
  Delay765/1 -> Delay769/1, Relational280/1
  Relational287/1 -> Delay792/1
  Delay701/1 -> Mux292/2
  Mux271/1 -> AddSub273/1, Delay760/1
  Mux277/1 -> AddSub279/1, Delay777/1
  Relational301/1 -> Delay727/1
  logi_b111/1 -> Relational265/2, Relational264/2
  Delay697/1 -> Mux207/2
  Delay711/1 -> Mux259/1
  Relational288/1 -> Delay795/1
  Delay817/1 -> Delay820/1, Relational271/1
  Delay659/1 -> Mux255/2
  Delay739/1 -> Delay741/1, Relational206/1
  Delay803/1 -> Mux289/2
  Relational295/1 -> Delay706/1
  Delay712/1 -> Mux259/2
  AddSub297/1 -> Mux296/3
  Mux254/1 -> AddSub255/1, Delay659/1
  Delay614/1 -> Mux237/2
  Relational253/1 -> Delay624/1
  AddSub256/1 -> Mux256/3
  Delay764/1 -> Delay765/1, Relational279/1
  Delay713/1 -> Mux280/2
  Delay780/1 -> Relational265/1, Delay689/1
  Delay660/1 -> Relational261/1, Delay635/1
  Mux260/1 -> AddSub262/1, Delay782/1
  Mux290/1 -> AddSub289/1, Delay743/1
  Relational286/1 -> Delay787/1
  AddSub283/1 -> Mux285/3
  Mux300/1 -> AddSub238/1, Delay612/1
  Delay679/1 -> Relational253/1, Delay682/1
  AddSub285/1 -> Mux286/3
  Delay807/1 -> Mux266/2
  Delay798/1 -> Mux288/1
  Delay684/1 -> Mux282/1
  Relational302/1 -> Delay720/1
  Delay762/1 -> Mux274/1
  Relational268/1 -> Delay809/1
  Delay703/1 -> Mux280/1
  AddSub272/1 -> Mux271/3
  Delay812/1 -> Delay814/1, Relational269/1
  Mux205/1 -> AddSub209/1, Delay753/1
  Delay821/1 -> Mux281/1
  AddSub254/1 -> Mux254/3
  Mux206/1 -> AddSub280/1, Delay779/1
  Relational277/1 -> Delay759/1
  Relational284/1 -> Delay784/1
  AddSub277/1 -> Mux277/3
  Delay775/1 -> Relational262/1, Delay780/1
  Delay444/1 -> Relational139/1, Delay617/1
  AddSub289/1 -> Mux298/3
  Mux259/1 -> AddSub293/1, Delay717/1
  Mux249/1 -> AddSub257/1, Delay640/1
  Delay799/1 -> Mux288/2
  logi_b119/1 -> Relational291/2, Relational293/2
  Relational278/1 -> Delay762/1
  Delay742/1 -> Mux298/1
  AddSub294/1 -> Mux299/3
  Relational208/1 -> Delay749/1
  Relational291/1 -> Delay704/1
  Delay640/1 -> Mux257/2
  Relational275/1 -> Delay755/1
  Delay719/1 -> Relational301/1, Delay739/1
  Mux257/1 -> Delay757/1, AddSub272/1
  Delay749/1 -> Mux205/1
  AddSub273/1 -> Mux273/3
  Delay741/1 -> Delay744/1, Relational207/1
  Delay796/1 -> Mux287/2
  logi_b103/1 -> Relational276/2, Relational282/2
  AddSub211/1 -> Mux260/3
  logi_b113/1 -> Relational267/2, Relational284/2
  Delay804/1 -> Mux265/2
  AddSub284/1 -> Mux282/3
  Delay776/1 -> Mux278/1
  Delay797/1 -> Relational290/1, Delay801/1
  Relational204/1 -> Delay677/1
  Delay681/1 -> Mux248/2
  AddSub274/1 -> Mux274/3
  AddSub268/1 -> Mux268/3
  Delay766/1 -> Mux275/1
  Relational260/1 -> Delay639/1
  AddSub257/1 -> Mux257/3
  AddSub275/1 -> Mux275/3
  Relational298/1 -> Delay732/1
  Delay781/1 -> Mux271/1
  Delay770/1 -> Mux276/1
  Delay746/1 -> Mux204/1
  Delay738/1 -> Relational239/1
  Relational300/1 -> Delay715/1
  Delay743/1 -> Mux298/2
  Relational266/1 -> Delay690/1
  Delay748/1 -> Relational210/1, Delay751/1
  Delay677/1 -> Mux247/1
  Mux276/1 -> AddSub277/1, Delay774/1
  Mux269/1 -> AddSub282/1, Delay823/1
  Delay801/1 -> Relational293/1, Delay699/1
  Relational297/1 -> Delay710/1
  Mux248/1 -> AddSub252/1, Delay625/1
  Delay754/1 -> Relational264/1, Delay693/1
  Relational265/1 -> Delay686/1
  Delay769/1 -> Delay772/1, Relational281/1
  Delay777/1 -> Mux278/2
  Delay612/1 -> Mux238/2
  Mux207/1 -> Delay688/1, AddSub264/1
  Mux289/1 -> AddSub291/1, Delay701/1
  Delay824/1 -> Relational291/1, Delay702/1
  logi_b117/1 -> Relational271/2, Relational289/2
  Mux293/1 -> AddSub296/1, Delay729/1
  logi_b108/1 -> Relational281/2, Relational208/2
  Mux280/1 -> AddSub278/1, Delay731/1
  Mux285/1 -> AddSub285/1, Delay793/1
  Delay639/1 -> Mux257/1
  AddSub265/1 -> Mux265/3
  logi_b116/1 -> Relational270/2, Relational288/2
  Mux288/1 -> AddSub288/1, Delay803/1
  AddSub276/1 -> Mux276/3
  Delay802/1 -> Mux289/1
  Delay720/1 -> Mux299/1
  Delay706/1 -> Mux293/1
  Relational207/1 -> Delay746/1
  Delay725/1 -> Mux300/2
  Delay686/1 -> Mux264/1
  Mux295/1 -> AddSub297/1, Delay734/1
  Delay699/1 -> Relational294/1, Delay714/1
  Delay727/1 -> Mux290/1
  Delay795/1 -> Mux287/1
  Relational239/1 -> Delay613/1
  Mux267/1 -> AddSub268/1, Delay816/1
  Delay759/1 -> Mux273/1
  Delay611/1 -> Mux238/1
  Delay773/1 -> Mux277/1
  AddSub236/1 -> Mux237/3
  AddSub255/1 -> Mux255/3
  Delay744/1 -> Delay748/1, Relational208/1
  Delay779/1 -> Mux279/2
  Mux298/1 -> AddSub299/1, Delay747/1
  logi_b124/1 -> Relational239/2, Relational238/2
  Relational280/1 -> Delay770/1
  Delay638/1 -> Delay758/1, Relational276/1
  Delay694/1 -> Mux262/1
  Delay689/1 -> Delay805/1, Relational266/1
  Delay808/1 -> Relational268/1, Delay812/1
  Mux296/1 -> AddSub298/1, Delay737/1
  Mux255/1 -> AddSub256/1, Delay662/1
  AddSub206/1 -> Mux205/3
  Delay693/1 -> Delay783/1, Relational272/1
  Delay695/1 -> Relational292/1, Delay719/1
  Delay793/1 -> Mux286/2
  Delay768/1 -> Mux275/2
  Relational282/1 -> Delay813/1
  Delay755/1 -> Mux279/1
  Delay792/1 -> Mux286/1
  Delay683/1 -> Mux270/2
  Delay655/1 -> Mux254/1
  Mux279/1 -> Delay692/1, AddSub211/1
  Delay710/1 -> Mux295/1
  Delay757/1 -> Mux271/2
  Delay637/1 -> Mux258/2
  Mux247/1 -> AddSub250/1, Delay681/1
  Delay784/1 -> Mux284/1
  Delay690/1 -> Mux265/1
  Mux265/1 -> AddSub266/1, Delay807/1
  AddSub266/1 -> Mux266/3
  Mux299/1 -> AddSub205/1, Delay725/1
  AddSub296/1 -> Mux295/3
  Delay815/1 -> Mux268/1
  logi_b123/1 -> Relational299/2, Relational205/2
  Relational258/1 -> Delay658/1
  Relational267/1 -> Delay806/1
  Relational279/1 -> Delay766/1
  AddSub290/1 -> Mux291/3
  Delay729/1 -> Mux295/2
  Delay731/1 -> Mux290/2
  Delay806/1 -> Mux266/1
  Delay692/1 -> Mux260/2
  logi_b122/1 -> Relational298/2, Relational302/2
  Mux278/1 -> AddSub210/1, Delay697/1
  AddSub280/1 -> Mux279/3
  Delay636/1 -> Mux258/1
  Relational270/1 -> Delay818/1
  Relational281/1 -> Delay773/1
  Relational269/1 -> Delay815/1
  AddSub271/1 -> Mux280/3
  AddSub258/1 -> Mux258/3
  Mux264/1 -> AddSub265/1, Delay804/1
  AddSub295/1 -> Mux293/3
  Relational294/1 -> Delay711/1
  Delay818/1 -> Mux269/1
  Delay702/1 -> Relational295/1, Delay709/1
  Delay810/1 -> Mux267/2
  logi_b107/1 -> Relational280/2, Relational207/2
  AddSub207/1 -> Mux259/3
  Delay685/1 -> Mux282/2
  Relational205/1 -> Delay724/1
  Delay750/1 -> Mux205/2
  logi_b114/1 -> Relational268/2, Relational286/2
  Delay732/1 -> Mux296/1
  Delay678/1 -> Mux247/2
  Relational261/1 -> Delay636/1
  Mux275/1 -> AddSub276/1, Delay771/1
  Relational273/1 -> Delay684/1
  Delay820/1 -> Relational273/1, Delay824/1
  Delay635/1 -> Delay695/1, Relational282/1
  Mux266/1 -> AddSub267/1, Delay810/1
  logi_b100/1 -> Relational250/2, Relational258/2
  AddSub287/1 -> Mux288/3
  Mux274/1 -> AddSub275/1, Delay768/1
  Delay783/1 -> Relational284/1, Delay786/1
  AddSub261/1 -> Mux270/3
  Delay691/1 -> Mux260/1
  Delay823/1 -> Mux281/2
  Delay819/1 -> Mux269/2
  Relational299/1 -> Delay736/1
  AddSub279/1 -> Mux278/3
  Delay752/1 -> Mux206/1
  Delay682/1 -> Relational260/1, Delay638/1
  Relational289/1 -> Delay798/1
  Delay656/1 -> Mux254/2
  AddSub286/1 -> Mux287/3
  Delay717/1 -> Mux263/2
  Mux262/1 -> AddSub263/1, Delay785/1
  Mux273/1 -> AddSub274/1, Delay763/1
  logi_b101/1 -> Relational253/2, Relational259/2
  Delay722/1 -> Relational205/1, Delay726/1
  Relational250/1 -> Delay680/1
  Delay774/1 -> Mux277/2
  logi_b104/1 -> Relational277/2, Relational292/2
  Mux282/1 -> AddSub290/1, Delay705/1
  AddSub293/1 -> Mux263/3
  Delay709/1 -> Delay730/1, Relational297/1
  Delay805/1 -> Relational267/1, Delay808/1
  Delay786/1 -> Relational286/1, Delay790/1
  Relational271/1 -> Delay821/1
  AddSub209/1 -> Mux206/3
  AddSub298/1 -> Mux297/3
  Delay714/1 -> Delay718/1, Relational300/1
  logi_b102/1 -> Relational260/2, Relational261/2
  AddSub210/1 -> Mux207/3
  Delay661/1 -> Mux256/1
  Mux268/1 -> AddSub269/1, Delay819/1
  AddSub252/1 -> Mux249/3
  Delay736/1 -> Mux297/1
  Delay708/1 -> Mux293/2
  Mux270/1 -> AddSub271/1, Delay713/1
  AddSub278/1 -> Mux290/3
  Mux292/1 -> Delay712/1, AddSub207/1
  Relational276/1 -> Delay781/1
  Delay751/1 -> Relational275/1, Delay754/1
  Delay730/1 -> Relational298/1, Delay735/1
  Delay688/1 -> Mux264/2
  Delay794/1 -> Delay797/1, Relational289/1
  Delay790/1 -> Delay791/1, Relational287/1
  logi_b118/1 -> Relational273/2, Relational290/2
  Delay809/1 -> Mux267/1
  Delay753/1 -> Mux206/2
  Relational262/1 -> Delay696/1
  Mux287/1 -> AddSub287/1, Delay799/1
  Delay782/1 -> Mux262/2
  Delay761/1 -> Relational278/1, Delay764/1
  Mux256/1 -> AddSub258/1, Delay637/1
  Relational293/1 -> Delay700/1
  Mux297/1 -> AddSub236/1, Delay614/1
  Mux284/1 -> AddSub283/1, Delay788/1
  Mux291/1 -> Delay708/1, AddSub295/1
  Delay813/1 -> Mux270/1
  logi_b106/1 -> Relational279/2, Relational206/2
  Delay772/1 -> Relational283/1, Delay775/1
  Delay791/1 -> Delay794/1, Relational288/1
  AddSub238/1 -> Mux238/3
  AddSub263/1 -> Mux284/3
  logi_b112/1 -> Relational266/2, Relational272/2
  Delay696/1 -> Mux207/1
  Relational272/1 -> Delay694/1
  Delay680/1 -> Mux248/1
  Relational210/1 -> Delay752/1
  Delay657/1 -> Relational259/1, Delay660/1
  Delay771/1 -> Mux276/2
  Relational238/1 -> Delay611/1
  Delay724/1 -> Mux300/1
  Delay816/1 -> Mux268/2
  Delay735/1 -> Relational299/1, Delay738/1
  Mux237/1 -> Slice1/1
  Mux138/1 -> AddSub254/1, Delay656/1
  logi_b99/1 -> Relational204/2, Relational203/2
  Mux137/1 -> AddSub249/1, Delay678/1
  Mux238/1 -> Slice/1
  Gate_out1/1 -> Output/1
  Constant5/1 -> Delay604/1
  Delay604/1 -> AddSub22/2
  Slice/1 -> Delay60/1, AddSub18/1, Delay59/1
  Delay610/1 -> Relational203/1, Delay615/1
  Delay615/1 -> Relational258/1, Delay657/1
  Delay616/1 -> Relational250/1, Delay679/1
  Delay617/1 -> Relational204/1, Delay616/1
  ROM2/1 -> Concat/2
  ROM3/1 -> Concat/3
  ROM4/1 -> Concat/4
  ROM1/1 -> Concat/1
  ROM7/1 -> Concat/7
  Concat/1 -> Scaling/1
  ROM5/1 -> Concat/5
  ROM6/1 -> Concat/6
  ROM8/1 -> Concat/8
  ROM10/1 -> Concat/10
  ROM11/1 -> Concat/11
  ROM9/1 -> Concat/9
  ROM14/1 -> Concat/14
  ROM13/1 -> Concat/13
  ROM15/1 -> Concat/15
  ROM12/1 -> Concat/12
  ROM16/1 -> Concat/16
  ROM22/1 -> Concat/22
  ROM32/1 -> Concat/32
  ROM31/1 -> Concat/31
  ROM26/1 -> Concat/26
  ROM30/1 -> Concat/30
  Slice3/1 -> ROM31/1, ROM32/1, ROM30/1, ROM29/1, ROM28/1, ROM27/1, ROM26/1, ROM25/1, ROM24/1, ROM23/1, ROM22/1, ROM21/1, ROM20/1, ROM19/1, ROM18/1, ROM17/1, ROM16/1, ROM15/1, ROM14/1, ROM13/1, ROM12/1, ROM11/1, ROM10/1, ROM9/1, ROM4/1, ROM1/1, ROM2/1, ROM3/1, ROM5/1, ROM6/1, ROM7/1, ROM8/1
  ROM29/1 -> Concat/29
  ROM27/1 -> Concat/27
  ROM21/1 -> Concat/21
  ROM20/1 -> Concat/20
  ROM23/1 -> Concat/23
  ROM25/1 -> Concat/25
  ROM17/1 -> Concat/17
  ROM28/1 -> Concat/28
  ROM19/1 -> Concat/19
  ROM18/1 -> Concat/18
  ROM24/1 -> Concat/24
  Slice1/1 -> Delay61/1
